simulink model "Boeing787_debug"  (R2015b)
(part 6 of 17)

      |             fcn1  = 'u(1)/39.37008' ;
      |         case 'Feet'
      |             name1 = 'ft/' ;
      |             fcn1  = 'u(1)/3.28084';
      |         case 'Yards'
      |             name1 = 'yd/' ;
      |             fcn1  = 'u(1)*3/3.28084' ;
      |         case 'Miles'
      |             name1 = 'mi/' ;
      |             fcn1  = 'u(1)*1609.344' ;
      |         case 'Nautical Miles'
      |             name1 = 'nmi/' ;
      |             fcn1  = 'u(1)*1852' ;
      |     end
      |     switch value2
      |         case 'Millisecond'
      |             name2 = 'ms' ;
      |             fcn2  = '*1000'  ;
      |         case 'Second'
      |             name2 = 's' ;
      |             fcn2  = '' ;
      |         case 'Minute'
      |             name2 = 'min' ;
      |             fcn2  = '/60' ;
      |         case 'Hour'
      |             name2 = 'hr' ;
      |             fcn2  = '/3600' ;
      |     end
      |     switch value3
      |         case 'Millimeters'
      |             name3 = 'mm/' ;
      |             fcn3  = '*1000' ;
      |         case 'Meters'
      |             name3 = 'm/' ;
      |             fcn3  = '' ;
      |         case 'Kilometers'
      |             name3 = 'km/' ;
      |             fcn3  = '/1000' ;
      |         case 'Inches'
      |             name3 = 'in/' ;
      |             fcn3  = '*39.37008' ;
      |         case 'Feet'
      |             name3 = 'ft/' ;
      |             fcn3  = '*3.28084';
      |         case 'Yards'
      |             name3 = 'yd/' ;
      |             fcn3  = '/3*3.28084' ;
      |         case 'Miles'
      |             name3 = 'mi/' ;
      |             fcn3  = '/1609.344' ;
      |         case 'Nautical Miles'
      |             name3 = 'nmi/' ;
      |             fcn3  = '/1852' ;
      |     end
      |     switch value4
      |         case 'Millisecond'
      |             name4 = 'ms' ;
      |             fcn4  = '/1000'  ;
      |         case 'Second'
      |             name4 = 's' ;
      |             fcn4  = '' ;
      |         case 'Minute'
      |             name4 = 'min' ;
      |             fcn4  = '*60' ;
      |         case 'Hour'
      |             name4 = 'hr' ;
      |             fcn4  = '*3600' ;
      |     end
      |     expr = [fcn1 fcn2 fcn3 fcn4] ;
      |     %set_param(blk,'func',func) ;
      |     set_param([blk '/conv_fcn'],'expr',expr) ;
      |     str1 = ['% this block of text is updated via dialog callbacks'];
      |     str2 = [char(39) 'horizontalAlignment' char(39) ',' char(39) 'center' char(39) ',' char(39) 'texmode' char(39) ',' char(39) 'on' char(39)] ;
      |     name = [char(39) name1 name2 ' to ' name3 name4 char(39)] ;
      |     str = sprintf('%s\ntext(.5,.5,%s,%s)',str1,name,str2) ;
      |     set_param(blk,'MaskDisplay',str) ;
      | end
      | clear blk value1 value2 value3 value4 expr name1 name2 name3 name4 name fcn1 fcn2 fcn3 fcn4 str1 str2 str
      mask TypeOptions totime: Millisecond | Second | Minute | Hour
      mask Callback totime:
      | blk = gcb ;
      | value1 = get_param(blk,'fromlen') ;
      | value2 = get_param(blk,'fromtime') ;
      | value3 = get_param(blk,'tolen') ;
      | value4 = get_param(blk,'totime') ;
      | if strcmp(get_param(blk,'vel'),'on')
      |     switch value1
      |         case 'Millimeters'
      |             name1 = 'mm/' ;
      |             fcn1  = 'u(1)/1000' ;
      |         case 'Meters'
      |             name1 = 'm/' ;
      |             fcn1  = 'u(1)' ;
      |         case 'Kilometers'
      |             name1 = 'km/' ;
      |             fcn1  = 'u(1)*1000' ;
      |         case 'Inches'
      |             name1 = 'in/' ;
      |             fcn1  = 'u(1)/39.37008' ;
      |         case 'Feet'
      |             name1 = 'ft/' ;
      |             fcn1  = 'u(1)/3.28084';
      |         case 'Yards'
      |             name1 = 'yd/' ;
      |             fcn1  = 'u(1)*3/3.28084' ;
      |         case 'Miles'
      |             name1 = 'mi/' ;
      |             fcn1  = 'u(1)*1609.344' ;
      |         case 'Nautical Miles'
      |             name1 = 'nmi/' ;
      |             fcn1  = 'u(1)*1852' ;
      |     end
      |     switch value2
      |         case 'Millisecond'
      |             name2 = 'ms' ;
      |             fcn2  = '*1000'  ;
      |         case 'Second'
      |             name2 = 's' ;
      |             fcn2  = '' ;
      |         case 'Minute'
      |             name2 = 'min' ;
      |             fcn2  = '/60' ;
      |         case 'Hour'
      |             name2 = 'hr' ;
      |             fcn2  = '/3600' ;
      |     end
      |     switch value3
      |         case 'Millimeters'
      |             name3 = 'mm/' ;
      |             fcn3  = '*1000' ;
      |         case 'Meters'
      |             name3 = 'm/' ;
      |             fcn3  = '' ;
      |         case 'Kilometers'
      |             name3 = 'km/' ;
      |             fcn3  = '/1000' ;
      |         case 'Inches'
      |             name3 = 'in/' ;
      |             fcn3  = '*39.37008' ;
      |         case 'Feet'
      |             name3 = 'ft/' ;
      |             fcn3  = '*3.28084';
      |         case 'Yards'
      |             name3 = 'yd/' ;
      |             fcn3  = '/3*3.28084' ;
      |         case 'Miles'
      |             name3 = 'mi/' ;
      |             fcn3  = '/1609.344' ;
      |         case 'Nautical Miles'
      |             name3 = 'nmi/' ;
      |             fcn3  = '/1852' ;
      |     end
      |     switch value4
      |         case 'Millisecond'
      |             name4 = 'ms' ;
      |             fcn4  = '/1000'  ;
      |         case 'Second'
      |             name4 = 's' ;
      |             fcn4  = '' ;
      |         case 'Minute'
      |             name4 = 'min' ;
      |             fcn4  = '*60' ;
      |         case 'Hour'
      |             name4 = 'hr' ;
      |             fcn4  = '*3600' ;
      |     end
      |     expr = [fcn1 fcn2 fcn3 fcn4] ;
      |     %set_param(blk,'func',func) ;
      |     set_param([blk '/conv_fcn'],'expr',expr) ;
      |     str1 = ['% this block of text is updated via dialog callbacks'];
      |     str2 = [char(39) 'horizontalAlignment' char(39) ',' char(39) 'center' char(39) ',' char(39) 'texmode' char(39) ',' char(39) 'on' char(39)] ;
      |     name = [char(39) name1 name2 ' to ' name3 name4 char(39)] ;
      |     str = sprintf('%s\ntext(.5,.5,%s,%s)',str1,name,str2) ;
      |     set_param(blk,'MaskDisplay',str) ;
      | end
      | clear blk value1 value2 value3 value4 expr name1 name2 name3 name4 name fcn1 fcn2 fcn3 fcn4 str1 str2 str
      mask Callback flow_rate:
      | blk = gcb ;
      | value = get_param(blk,'flow_rate') ;
      | cellarr = get_param(blk,'MaskVisibilities') ;
      | ind = [1 4 9 12 15 18 21 24 27 30 33 38 43] ;
      | if strcmp(value,'on')
      |     cellarr(ind) = {'off'} ; cellarr(38:42) = {'on'} ;
      |     value1 = get_param(blk,'fromflowvol') ;
      |     value2 = get_param(blk,'fromflvoltime') ;
      |     value3 = get_param(blk,'toflowvol') ;
      |     value4 = get_param(blk,'toflvoltime') ;
      |     if strcmp(get_param(blk,'flow_rate'),'on')
      |         switch value1
      |             case 'Milliliters'
      |                 name1 = 'mL/' ;
      |                 fcn1  = 'u(1)*(1e-6)' ;
      |             case 'Liters'
      |                 name1 = 'L/' ;
      |                 fcn1  = 'u(1)*.001' ;
      |             case 'Cubic Centimeters'
      |                 name1 = 'cm^3/' ;
      |                 fcn1  = 'u(1)*(1e-6)' ;
      |             case 'Cubic Meters'
      |                 name1 = 'm^3/' ;
      |                 fcn1  = 'u(1)' ;
      |             case 'Ounces'
      |                 name1 = 'oz/' ;
      |                 fcn1  = 'u(1)*(2.957353e-5)';
      |             case 'Gallons'
      |                 name1 = 'gal/' ;
      |                 fcn1  = 'u(1)*.00378541' ;
      |             case 'Cubic Inches'
      |                 name1 = 'in^3/' ;
      |                 fcn1  = 'u(1)*(1.6387e-5)' ;
      |             case 'Cubic Feet'
      |                 name1 = 'ft^3/' ;
      |                 fcn1  = 'u(1)*.0283168' ;
      |         end
      |         switch value2
      |             case 'Millisecond'
      |                 name2 = 'ms' ;
      |                 fcn2  = '*1000'  ;
      |             case 'Second'
      |                 name2 = 's' ;
      |                 fcn2  = '' ;
      |             case 'Minute'
      |                 name2 = 'min' ;
      |                 fcn2  = '/60' ;
      |             case 'Hour'
      |                 name2 = 'hr' ;
      |                 fcn2  = '/3600' ;
      |         end
      |         switch value3
      |             case 'Milliliters'
      |                 name3 = 'mL/' ;
      |                 fcn3  = '/(1e-6)' ;
      |             case 'Liters'
      |                 name3 = 'L/' ;
      |                 fcn3  = '/.001' ;
      |             case 'Cubic Centimeters'
      |                 name3 = 'cm^3/' ;
      |                 fcn3  = '/(1e-6)' ;
      |             case 'Cubic Meters'
      |                 name3 = 'm^3/' ;
      |                 fcn3  = '' ;
      |             case 'Ounces'
      |                 name3 = 'oz/' ;
      |                 fcn3  = '/(2.957353e-5)';
      |             case 'Gallons'
      |                 name3 = 'gal/' ;
      |                 fcn3  = '/.00378541' ;
      |             case 'Cubic Inches'
      |                 name3 = 'in^3/' ;
      |                 fcn3  = '/(1.6387e-5)' ;
      |             case 'Cubic Feet'
      |                 name3 = 'ft^3/' ;
      |                 fcn3  = '/.0283168' ;
      |         end
      |         switch value4
      |             case 'Millisecond'
      |                 name4 = 'ms' ;
      |                 fcn4  = '/1000'  ;
      |             case 'Second'
      |                 name4 = 's' ;
      |                 fcn4  = '' ;
      |             case 'Minute'
      |                 name4 = 'min' ;
      |                 fcn4  = '*60' ;
      |             case 'Hour'
      |                 name4 = 'hr' ;
      |                 fcn4  = '*3600' ;
      |         end
      |         expr = [fcn1 fcn2 fcn3 fcn4] ;
      |         %set_param(blk,'func',func) ;
      |         set_param([blk '/conv_fcn'],'expr',expr) ;
      |         str1 = ['% this block of text is updated via dialog callbacks'];
      |         str2 = [char(39) 'horizontalAlignment' char(39) ',' char(39) 'center' char(39) ',' char(39) 'texmode' char(39) ',' char(39) 'on' char(39)] ;
      |         name = [char(39) name1 name2 ' to ' name3 name4 char(39)] ;
      |         str = sprintf('%s\ntext(.5,.5,%s,%s)',str1,name,str2) ;
      |         set_param(blk,'MaskDisplay',str) ;
      |     end
      |     clear value1 value2 value3 value4 expr name1 name2 name3 name4 name fcn1 fcn2 fcn3 fcn4 str1 str2 str
      | else
      |     cellarr(39:42) = {'off'} ; val = get_param(blk,'MaskValues') ;
      |     for i=1:length(ind)
      |         a = findstr(val{ind(i)},'on') ;
      |         b(i) = isempty(a) ;
      |     end
      |     if isempty(find(b==0)) ;
      |         cellarr(ind) = {'on'} ;
      |     end
      | end
      | set_param(blk,'MaskVisibilities',cellarr) ;
      | clear blk value cellarr ind a b val i
      mask TypeOptions fromflowvol: Milliliters | Liters | Cubic Centimeters | Cubic Meters | Ounces | Gallons | Cubic Inches | Cubic Feet
      mask Callback fromflowvol:
      | blk = gcb ;
      | value1 = get_param(blk,'fromflowvol') ;
      | value2 = get_param(blk,'fromflvoltime') ;
      | value3 = get_param(blk,'toflowvol') ;
      | value4 = get_param(blk,'toflvoltime') ;
      | if strcmp(get_param(blk,'flow_rate'),'on')
      |     switch value1
      |         case 'Milliliters'
      |             name1 = 'mL/' ;
      |             fcn1  = 'u(1)*(1e-6)';
      |         case 'Liters'
      |             name1 = 'L/' ;
      |             fcn1  = 'u(1)*.001' ;
      |         case 'Cubic Centimeters'
      |             name1 = 'cm^3/' ;
      |             fcn1  = 'u(1)*(1e-6)' ;
      |         case 'Cubic Meters'
      |             name1 = 'm^3/' ;
      |             fcn1  = 'u(1)' ;
      |         case 'Ounces'
      |             name1 = 'oz/' ;
      |             fcn1  = 'u(1)*(2.957353e-5)';
      |         case 'Gallons'
      |             name1 = 'gal/' ;
      |             fcn1  = 'u(1)*.00378541' ;
      |         case 'Cubic Inches'
      |             name1 = 'in^3/' ;
      |             fcn1  = 'u(1)*(1.6387e-5)' ;
      |         case 'Cubic Feet'
      |             name1 = 'ft^3/' ;
      |             fcn1  = 'u(1)*.0283168' ;
      |     end
      |     switch value2
      |         case 'Millisecond'
      |             name2 = 'ms' ;
      |             fcn2  = '*1000'  ;
      |         case 'Second'
      |             name2 = 's' ;
      |             fcn2  = '' ;
      |         case 'Minute'
      |             name2 = 'min' ;
      |             fcn2  = '/60' ;
      |         case 'Hour'
      |             name2 = 'hr' ;
      |             fcn2  = '/3600' ;
      |     end
      |     switch value3
      |         case 'Milliliters'
      |             name3 = 'mL/' ;
      |             fcn3  = '/(1e-6)' ;
      |         case 'Liters'
      |             name3 = 'L/' ;
      |             fcn3  = '/.001' ;
      |         case 'Cubic Centimeters'
      |             name3 = 'cm^3/' ;
      |             fcn3  = '/(1e-6)' ;
      |         case 'Cubic Meters'
      |             name3 = 'm^3/' ;
      |             fcn3  = '' ;
      |         case 'Ounces'
      |             name3 = 'oz/' ;
      |             fcn3  = '/(2.957353e-5)';
      |         case 'Gallons'
      |             name3 = 'gal/' ;
      |             fcn3  = '/.00378541' ;
      |         case 'Cubic Inches'
      |             name3 = 'in^3/' ;
      |             fcn3  = '/(1.6387e-5)' ;
      |         case 'Cubic Feet'
      |             name3 = 'ft^3/' ;
      |             fcn3  = '/.0283168' ;
      |     end
      |     switch value4
      |         case 'Millisecond'
      |             name4 = 'ms' ;
      |             fcn4  = '/1000'  ;
      |         case 'Second'
      |             name4 = 's' ;
      |             fcn4  = '' ;
      |         case 'Minute'
      |             name4 = 'min' ;
      |             fcn4  = '*60' ;
      |         case 'Hour'
      |             name4 = 'hr' ;
      |             fcn4  = '*3600' ;
      |     end
      |     expr = [fcn1 fcn2 fcn3 fcn4] ;
      |     %set_param(blk,'func',func) ;
      |     set_param([blk '/conv_fcn'],'expr',expr) ;
      |     str1 = ['% this block of text is updated via dialog callbacks'];
      |     str2 = [char(39) 'horizontalAlignment' char(39) ',' char(39) 'center' char(39) ',' char(39) 'texmode' char(39) ',' char(39) 'on' char(39)] ;
      |     name = [char(39) name1 name2 ' to ' name3 name4 char(39)] ;
      |     str = sprintf('%s\ntext(.5,.5,%s,%s)',str1,name,str2) ;
      |     set_param(blk,'MaskDisplay',str) ;
      | end
      | clear blk value1 value2 value3 value4 expr name1 name2 name3 name4 name fcn1 fcn2 fcn3 fcn4 str1 str2 str
      mask TypeOptions fromflvoltime: Millisecond | Second | Minute | Hour
      mask Callback fromflvoltime:
      | blk = gcb ;
      | value1 = get_param(blk,'fromflowvol') ;
      | value2 = get_param(blk,'fromflvoltime') ;
      | value3 = get_param(blk,'toflowvol') ;
      | value4 = get_param(blk,'toflvoltime') ;
      | if strcmp(get_param(blk,'flow_rate'),'on')
      |     switch value1
      |         case 'Milliliters'
      |             name1 = 'mL/' ;
      |             fcn1  = 'u(1)*(1e-6)' ;
      |         case 'Liters'
      |             name1 = 'L/' ;
      |             fcn1  = 'u(1)*.001' ;
      |         case 'Cubic Centimeters'
      |             name1 = 'cm^3/' ;
      |             fcn1  = 'u(1)*(1e-6)' ;
      |         case 'Cubic Meters'
      |             name1 = 'm^3/' ;
      |             fcn1  = 'u(1)' ;
      |         case 'Ounces'
      |             name1 = 'oz/' ;
      |             fcn1  = 'u(1)*(2.957353e-5)';
      |         case 'Gallons'
      |             name1 = 'gal/' ;
      |             fcn1  = 'u(1)*.00378541' ;
      |         case 'Cubic Inches'
      |             name1 = 'in^3/' ;
      |             fcn1  = 'u(1)*(1.6387e-5)' ;
      |         case 'Cubic Feet'
      |             name1 = 'ft^3/' ;
      |             fcn1  = 'u(1)*.0283168' ;
      |     end
      |     switch value2
      |         case 'Millisecond'
      |             name2 = 'ms' ;
      |             fcn2  = '*1000'  ;
      |         case 'Second'
      |             name2 = 's' ;
      |             fcn2  = '' ;
      |         case 'Minute'
      |             name2 = 'min' ;
      |             fcn2  = '/60' ;
      |         case 'Hour'
      |             name2 = 'hr' ;
      |             fcn2  = '/3600' ;
      |     end
      |     switch value3
      |         case 'Milliliters'
      |             name3 = 'mL/' ;
      |             fcn3  = '/(1e-6)' ;
      |         case 'Liters'
      |             name3 = 'L/' ;
      |             fcn3  = '/.001' ;
      |         case 'Cubic Centimeters'
      |             name3 = 'cm^3/' ;
      |             fcn3  = '/(1e-6)' ;
      |         case 'Cubic Meters'
      |             name3 = 'm^3/' ;
      |             fcn3  = '' ;
      |         case 'Ounces'
      |             name3 = 'oz/' ;
      |             fcn3  = '/(2.957353e-5)';
      |         case 'Gallons'
      |             name3 = 'gal/' ;
      |             fcn3  = '/.00378541' ;
      |         case 'Cubic Inches'
      |             name3 = 'in^3/' ;
      |             fcn3  = '/(1.6387e-5)' ;
      |         case 'Cubic Feet'
      |             name3 = 'ft^3/' ;
      |             fcn3  = '/.0283168' ;
      |     end
      |     switch value4
      |         case 'Millisecond'
      |             name4 = 'ms' ;
      |             fcn4  = '/1000'  ;
      |         case 'Second'
      |             name4 = 's' ;
      |             fcn4  = '' ;
      |         case 'Minute'
      |             name4 = 'min' ;
      |             fcn4  = '*60' ;
      |         case 'Hour'
      |             name4 = 'hr' ;
      |             fcn4  = '*3600' ;
      |     end
      |     expr = [fcn1 fcn2 fcn3 fcn4] ;
      |     %set_param(blk,'func',func) ;
      |     set_param([blk '/conv_fcn'],'expr',expr) ;
      |     str1 = ['% this block of text is updated via dialog callbacks'];
      |     str2 = [char(39) 'horizontalAlignment' char(39) ',' char(39) 'center' char(39) ',' char(39) 'texmode' char(39) ',' char(39) 'on' char(39)] ;
      |     name = [char(39) name1 name2 ' to ' name3 name4 char(39)] ;
      |     str = sprintf('%s\ntext(.5,.5,%s,%s)',str1,name,str2) ;
      |     set_param(blk,'MaskDisplay',str) ;
      | end
      | clear blk value1 value2 value3 value4 expr name1 name2 name3 name4 name fcn1 fcn2 fcn3 fcn4 str1 str2 str
      mask TypeOptions toflowvol: Milliliters | Liters | Cubic Centimeters | Cubic Meters | Ounces | Gallons | Cubic Inches | Cubic Feet
      mask Callback toflowvol:
      | blk = gcb ;
      | value1 = get_param(blk,'fromflowvol') ;
      | value2 = get_param(blk,'fromflvoltime') ;
      | value3 = get_param(blk,'toflowvol') ;
      | value4 = get_param(blk,'toflvoltime') ;
      | if strcmp(get_param(blk,'flow_rate'),'on')
      |     switch value1
      |         case 'Milliliters'
      |             name1 = 'mL/' ;
      |             fcn1  = 'u(1)*(1e-6)' ;
      |         case 'Liters'
      |             name1 = 'L/' ;
      |             fcn1  = 'u(1)*.001' ;
      |         case 'Cubic Centimeters'
      |             name1 = 'cm^3/' ;
      |             fcn1  = 'u(1)*(1e-6)' ;
      |         case 'Cubic Meters'
      |             name1 = 'm^3/' ;
      |             fcn1  = 'u(1)' ;
      |         case 'Ounces'
      |             name1 = 'oz/' ;
      |             fcn1  = 'u(1)*(2.957353e-5)';
      |         case 'Gallons'
      |             name1 = 'gal/' ;
      |             fcn1  = 'u(1)*.00378541' ;
      |         case 'Cubic Inches'
      |             name1 = 'in^3/' ;
      |             fcn1  = 'u(1)*(1.6387e-5)' ;
      |         case 'Cubic Feet'
      |             name1 = 'ft^3/' ;
      |             fcn1  = 'u(1)*.0283168' ;
      |     end
      |     switch value2
      |         case 'Millisecond'
      |             name2 = 'ms' ;
      |             fcn2  = '*1000'  ;
      |         case 'Second'
      |             name2 = 's' ;
      |             fcn2  = '' ;
      |         case 'Minute'
      |             name2 = 'min' ;
      |             fcn2  = '/60' ;
      |         case 'Hour'
      |             name2 = 'hr' ;
      |             fcn2  = '/3600' ;
      |     end
      |     switch value3
      |         case 'Milliliters'
      |             name3 = 'mL/' ;
      |             fcn3  = '/(1e-6)' ;
      |         case 'Liters'
      |             name3 = 'L/' ;
      |             fcn3  = '/.001' ;
      |         case 'Cubic Centimeters'
      |             name3 = 'cm^3/' ;
      |             fcn3  = '/(1e-6)' ;
      |         case 'Cubic Meters'
      |             name3 = 'm^3/' ;
      |             fcn3  = '' ;
      |         case 'Ounces'
      |             name3 = 'oz/' ;
      |             fcn3  = '/(2.957353e-5)';
      |         case 'Gallons'
      |             name3 = 'gal/' ;
      |             fcn3  = '/.00378541' ;
      |         case 'Cubic Inches'
      |             name3 = 'in^3/' ;
      |             fcn3  = '/(1.6387e-5)' ;
      |         case 'Cubic Feet'
      |             name3 = 'ft^3/' ;
      |             fcn3  = '/.0283168' ;
      |     end
      |     switch value4
      |         case 'Millisecond'
      |             name4 = 'ms' ;
      |             fcn4  = '/1000'  ;
      |         case 'Second'
      |             name4 = 's' ;
      |             fcn4  = '' ;
      |         case 'Minute'
      |             name4 = 'min' ;
      |             fcn4  = '*60' ;
      |         case 'Hour'
      |             name4 = 'hr' ;
      |             fcn4  = '*3600' ;
      |     end
      |     expr = [fcn1 fcn2 fcn3 fcn4] ;
      |     %set_param(blk,'func',func) ;
      |     set_param([blk '/conv_fcn'],'expr',expr) ;
      |     str1 = ['% this block of text is updated via dialog callbacks'];
      |     str2 = [char(39) 'horizontalAlignment' char(39) ',' char(39) 'center' char(39) ',' char(39) 'texmode' char(39) ',' char(39) 'on' char(39)] ;
      |     name = [char(39) name1 name2 ' to ' name3 name4 char(39)] ;
      |     str = sprintf('%s\ntext(.5,.5,%s,%s)',str1,name,str2) ;
      |     set_param(blk,'MaskDisplay',str) ;
      | end
      | clear blk value1 value2 value3 value4 expr name1 name2 name3 name4 name fcn1 fcn2 fcn3 fcn4 str1 str2 str
      mask TypeOptions toflvoltime: Millisecond | Second | Minute | Hour
      mask Callback toflvoltime:
      | blk = gcb ;
      | value1 = get_param(blk,'fromflowvol') ;
      | value2 = get_param(blk,'fromflvoltime') ;
      | value3 = get_param(blk,'toflowvol') ;
      | value4 = get_param(blk,'toflvoltime') ;
      | if strcmp(get_param(blk,'flow_rate'),'on')
      |     switch value1
      |         case 'Milliliters'
      |             name1 = 'mL/' ;
      |             fcn1  = 'u(1)*(1e-6)' ;
      |         case 'Liters'
      |             name1 = 'L/' ;
      |             fcn1  = 'u(1)*.001' ;
      |         case 'Cubic Centimeters'
      |             name1 = 'cm^3/' ;
      |             fcn1  = 'u(1)*(1e-6)' ;
      |         case 'Cubic Meters'
      |             name1 = 'm^3/' ;
      |             fcn1  = 'u(1)' ;
      |         case 'Ounces'
      |             name1 = 'oz/' ;
      |             fcn1  = 'u(1)*(2.957353e-5)';
      |         case 'Gallons'
      |             name1 = 'gal/' ;
      |             fcn1  = 'u(1)*.00378541' ;
      |         case 'Cubic Inches'
      |             name1 = 'in^3/' ;
      |             fcn1  = 'u(1)*(1.6387e-5)' ;
      |         case 'Cubic Feet'
      |             name1 = 'ft^3/' ;
      |             fcn1  = 'u(1)*.0283168' ;
      |     end
      |     switch value2
      |         case 'Millisecond'
      |             name2 = 'ms' ;
      |             fcn2  = '*1000'  ;
      |         case 'Second'
      |             name2 = 's' ;
      |             fcn2  = '' ;
      |         case 'Minute'
      |             name2 = 'min' ;
      |             fcn2  = '/60' ;
      |         case 'Hour'
      |             name2 = 'hr' ;
      |             fcn2  = '/3600' ;
      |     end
      |     switch value3
      |         case 'Milliliters'
      |             name3 = 'mL/' ;
      |             fcn3  = '/(1e-6)' ;
      |         case 'Liters'
      |             name3 = 'L/' ;
      |             fcn3  = '/.001' ;
      |         case 'Cubic Centimeters'
      |             name3 = 'cm^3/' ;
      |             fcn3  = '/(1e-6)' ;
      |         case 'Cubic Meters'
      |             name3 = 'm^3/' ;
      |             fcn3  = '' ;
      |         case 'Ounces'
      |             name3 = 'oz/' ;
      |             fcn3  = '/(2.957353e-5)';
      |         case 'Gallons'
      |             name3 = 'gal/' ;
      |             fcn3  = '/.00378541' ;
      |         case 'Cubic Inches'
      |             name3 = 'in^3/' ;
      |             fcn3  = '/(1.6387e-5)' ;
      |         case 'Cubic Feet'
      |             name3 = 'ft^3/' ;
      |             fcn3  = '/.0283168' ;
      |     end
      |     switch value4
      |         case 'Millisecond'
      |             name4 = 'ms' ;
      |             fcn4  = '/1000'  ;
      |         case 'Second'
      |             name4 = 's' ;
      |             fcn4  = '' ;
      |         case 'Minute'
      |             name4 = 'min' ;
      |             fcn4  = '*60' ;
      |         case 'Hour'
      |             name4 = 'hr' ;
      |             fcn4  = '*3600' ;
      |     end
      |     expr = [fcn1 fcn2 fcn3 fcn4] ;
      |     %set_param(blk,'func',func) ;
      |     set_param([blk '/conv_fcn'],'expr',expr) ;
      |     str1 = ['% this block of text is updated via dialog callbacks'];
      |     str2 = [char(39) 'horizontalAlignment' char(39) ',' char(39) 'center' char(39) ',' char(39) 'texmode' char(39) ',' char(39) 'on' char(39)] ;
      |     name = [char(39) name1 name2 ' to ' name3 name4 char(39)] ;
      |     str = sprintf('%s\ntext(.5,.5,%s,%s)',str1,name,str2) ;
      |     set_param(blk,'MaskDisplay',str) ;
      | end
      | clear blk value1 value2 value3 value4 expr name1 name2 name3 name4 name fcn1 fcn2 fcn3 fcn4 str1 str2 str
      mask Callback mfr:
      | blk = gcb ;
      | value = get_param(blk,'mfr') ;
      | cellarr = get_param(blk,'MaskVisibilities') ;
      | ind = [1 4 9 12 15 18 21 24 27 30 33 38 43] ;
      | if strcmp(value,'on')
      |     cellarr(ind) = {'off'} ; cellarr(43:47) = {'on'} ;
      |     value1 = get_param(blk,'frommfr') ;
      |     value2 = get_param(blk,'frommfrtime') ;
      |     value3 = get_param(blk,'tomfr') ;
      |     value4 = get_param(blk,'tomfrtime') ;
      |     if strcmp(get_param(blk,'mfr'),'on')
      |         switch value1
      |             case 'Grams'
      |                 name1 = 'g/' ;
      |                 fcn1  = 'u(1)*.001' ;
      |             case 'Kilograms'
      |                 name1 = 'kg/' ;
      |                 fcn1  = 'u(1)' ;
      |             case 'Ounces'
      |                 name1 = 'oz/' ;
      |                 fcn1  = 'u(1)*.45359237/16' ;
      |             case 'Pounds-Mass'
      |                 name1 = 'lbm/' ;
      |                 fcn1  = 'u(1)*.45359237' ;
      |             case 'Slugs'
      |                 name1 = 'slg/' ;
      |                 fcn1  = 'u(1)*14.5939';
      |         end
      |         switch value2
      |             case 'Millisecond'
      |                 name2 = 'ms' ;
      |                 fcn2  = '*1000'  ;
      |             case 'Second'
      |                 name2 = 's' ;
      |                 fcn2  = '' ;
      |             case 'Minute'
      |                 name2 = 'min' ;
      |                 fcn2  = '/60' ;
      |             case 'Hour'
      |                 name2 = 'hr' ;
      |                 fcn2  = '/3600' ;
      |         end
      |         switch value3
      |             case 'Grams'
      |                 name3 = 'g/' ;
      |                 fcn3  = '/.001' ;
      |             case 'Kilograms'
      |                 name3 = 'kg/' ;
      |                 fcn3  = '' ;
      |             case 'Ounces'
      |                 name3 = 'oz/' ;
      |                 fcn3  = '/.45359237*16' ;
      |             case 'Pounds-Mass'
      |                 name3 = 'lbm/' ;
      |                 fcn3  = '/.45359237' ;
      |             case 'Slugs'
      |                 name3 = 'slg/' ;
      |                 fcn3  = '/14.5939';
      |         end
      |         switch value4
      |             case 'Millisecond'
      |                 name4 = 'ms' ;
      |                 fcn4  = '/1000'  ;
      |             case 'Second'
      |                 name4 = 's' ;
      |                 fcn4  = '' ;
      |             case 'Minute'
      |                 name4 = 'min' ;
      |                 fcn4  = '*60' ;
      |             case 'Hour'
      |                 name4 = 'hr' ;
      |                 fcn4  = '*3600' ;
      |         end
      |         expr = [fcn1 fcn2 fcn3 fcn4] ;
      |         %set_param(blk,'func',func) ;
      |         set_param([blk '/conv_fcn'],'expr',expr) ;
      |         str1 = ['% this block of text is updated via dialog callbacks'];
      |         str2 = [char(39) 'horizontalAlignment' char(39) ',' char(39) 'center' char(39) ',' char(39) 'texmode' char(39) ',' char(39) 'on' char(39)] ;
      |         name = [char(39) name1 name2 ' to ' name3 name4 char(39)] ;
      |         str = sprintf('%s\ntext(.5,.5,%s,%s)',str1,name,str2) ;
      |         set_param(blk,'MaskDisplay',str) ;
      |     end
      |     clear value1 value2 value3 value4 expr name1 name2 name3 name4 name fcn1 fcn2 fcn3 fcn4 str1 str2 str
      | else
      |     cellarr(44:47) = {'off'} ; val = get_param(blk,'MaskValues') ;
      |     for i=1:length(ind)
      |         a = findstr(val{ind(i)},'on') ;
      |         b(i) = isempty(a) ;
      |     end
      |     if isempty(find(b==0)) ;
      |         cellarr(ind) = {'on'} ;
      |     end
      | end
      | set_param(blk,'MaskVisibilities',cellarr) ;
      | clear blk value cellarr ind a b val i
      mask TypeOptions frommfr: Grams | Kilograms | Ounces | Pounds-Mass | Slugs
      mask Callback frommfr:
      | blk = gcb ;
      | value1 = get_param(blk,'frommfr') ;
      | value2 = get_param(blk,'frommfrtime') ;
      | value3 = get_param(blk,'tomfr') ;
      | value4 = get_param(blk,'tomfrtime') ;
      | if strcmp(get_param(blk,'mfr'),'on')
      |     switch value1
      |         case 'Grams'
      |             name1 = 'g/' ;
      |             fcn1  = 'u(1)*.001' ;
      |         case 'Kilograms'
      |             name1 = 'kg/' ;
      |             fcn1  = 'u(1)' ;
      |         case 'Ounces'
      |             name1 = 'oz/' ;
      |             fcn1  = 'u(1)*.45359237/16' ;
      |         case 'Pounds-Mass'
      |             name1 = 'lbm/' ;
      |             fcn1  = 'u(1)*.45359237' ;
      |         case 'Slugs'
      |             name1 = 'slg/' ;
      |             fcn1  = 'u(1)*14.5939';
      |     end
      |     switch value2
      |         case 'Millisecond'
      |             name2 = 'ms' ;
      |             fcn2  = '*1000'  ;
      |         case 'Second'
      |             name2 = 's' ;
      |             fcn2  = '' ;
      |         case 'Minute'
      |             name2 = 'min' ;
      |             fcn2  = '/60' ;
      |         case 'Hour'
      |             name2 = 'hr' ;
      |             fcn2  = '/3600' ;
      |     end
      |     switch value3
      |         case 'Grams'
      |             name3 = 'g/' ;
      |             fcn3  = '/.001' ;
      |         case 'Kilograms'
      |             name3 = 'kg/' ;
      |             fcn3  = '' ;
      |         case 'Ounces'
      |             name3 = 'oz/' ;
      |             fcn3  = '/.45359237*16' ;
      |         case 'Pounds-Mass'
      |             name3 = 'lbm/' ;
      |             fcn3  = '/.45359237' ;
      |         case 'Slugs'
      |             name3 = 'slg/' ;
      |             fcn3  = '/14.5939';
      |     end
      |     switch value4
      |         case 'Millisecond'
      |             name4 = 'ms' ;
      |             fcn4  = '/1000'  ;
      |         case 'Second'
      |             name4 = 's' ;
      |             fcn4  = '' ;
      |         case 'Minute'
      |             name4 = 'min' ;
      |             fcn4  = '*60' ;
      |         case 'Hour'
      |             name4 = 'hr' ;
      |             fcn4  = '*3600' ;
      |     end
      |     expr = [fcn1 fcn2 fcn3 fcn4] ;
      |     %set_param(blk,'func',func) ;
      |     set_param([blk '/conv_fcn'],'expr',expr) ;
      |     str1 = ['% this block of text is updated via dialog callbacks'];
      |     str2 = [char(39) 'horizontalAlignment' char(39) ',' char(39) 'center' char(39) ',' char(39) 'texmode' char(39) ',' char(39) 'on' char(39)] ;
      |     name = [char(39) name1 name2 ' to ' name3 name4 char(39)] ;
      |     str = sprintf('%s\ntext(.5,.5,%s,%s)',str1,name,str2) ;
      |     set_param(blk,'MaskDisplay',str) ;
      | end
      | clear blk value1 value2 value3 value4 expr name1 name2 name3 name4 name fcn1 fcn2 fcn3 fcn4 str1 str2 str
      mask TypeOptions frommfrtime: Millisecond | Second | Minute | Hour
      mask Callback frommfrtime:
      | blk = gcb ;
      | value1 = get_param(blk,'frommfr') ;
      | value2 = get_param(blk,'frommfrtime') ;
      | value3 = get_param(blk,'tomfr') ;
      | value4 = get_param(blk,'tomfrtime') ;
      | if strcmp(get_param(blk,'mfr'),'on')
      |     switch value1
      |         case 'Grams'
      |             name1 = 'g/' ;
      |             fcn1  = 'u(1)*.001' ;
      |         case 'Kilograms'
      |             name1 = 'kg/' ;
      |             fcn1  = 'u(1)' ;
      |         case 'Ounces'
      |             name1 = 'oz/' ;
      |             fcn1  = 'u(1)*.45359237/16' ;
      |         case 'Pounds-Mass'
      |             name1 = 'lbm/' ;
      |             fcn1  = 'u(1)*.45359237' ;
      |         case 'Slugs'
      |             name1 = 'slg/' ;
      |             fcn1  = 'u(1)*14.5939';
      |     end
      |     switch value2
      |         case 'Millisecond'
      |             name2 = 'ms' ;
      |             fcn2  = '*1000'  ;
      |         case 'Second'
      |             name2 = 's' ;
      |             fcn2  = '' ;
      |         case 'Minute'
      |             name2 = 'min' ;
      |             fcn2  = '/60' ;
      |         case 'Hour'
      |             name2 = 'hr' ;
      |             fcn2  = '/3600' ;
      |     end
      |     switch value3
      |         case 'Grams'
      |             name3 = 'g/' ;
      |             fcn3  = '/.001' ;
      |         case 'Kilograms'
      |             name3 = 'kg/' ;
      |             fcn3  = '' ;
      |         case 'Ounces'
      |             name3 = 'oz/' ;
      |             fcn3  = '/.45359237*16' ;
      |         case 'Pounds-Mass'
      |             name3 = 'lbm/' ;
      |             fcn3  = '/.45359237' ;
      |         case 'Slugs'
      |             name3 = 'slg/' ;
      |             fcn3  = '/14.5939';
      |     end
      |     switch value4
      |         case 'Millisecond'
      |             name4 = 'ms' ;
      |             fcn4  = '/1000'  ;
      |         case 'Second'
      |             name4 = 's' ;
      |             fcn4  = '' ;
      |         case 'Minute'
      |             name4 = 'min' ;
      |             fcn4  = '*60' ;
      |         case 'Hour'
      |             name4 = 'hr' ;
      |             fcn4  = '*3600' ;
      |     end
      |     expr = [fcn1 fcn2 fcn3 fcn4] ;
      |     %set_param(blk,'func',func) ;
      |     set_param([blk '/conv_fcn'],'expr',expr) ;
      |     str1 = ['% this block of text is updated via dialog callbacks'];
      |     str2 = [char(39) 'horizontalAlignment' char(39) ',' char(39) 'center' char(39) ',' char(39) 'texmode' char(39) ',' char(39) 'on' char(39)] ;
      |     name = [char(39) name1 name2 ' to ' name3 name4 char(39)] ;
      |     str = sprintf('%s\ntext(.5,.5,%s,%s)',str1,name,str2) ;
      |     set_param(blk,'MaskDisplay',str) ;
      | end
      | clear blk value1 value2 value3 value4 expr name1 name2 name3 name4 name fcn1 fcn2 fcn3 fcn4 str1 str2 str
      mask TypeOptions tomfr: Grams | Kilograms | Ounces | Pounds-Mass | Slugs
      mask Callback tomfr:
      | blk = gcb ;
      | value1 = get_param(blk,'frommfr') ;
      | value2 = get_param(blk,'frommfrtime') ;
      | value3 = get_param(blk,'tomfr') ;
      | value4 = get_param(blk,'tomfrtime') ;
      | if strcmp(get_param(blk,'mfr'),'on')
      |     switch value1
      |         case 'Grams'
      |             name1 = 'g/' ;
      |             fcn1  = 'u(1)*.001' ;
      |         case 'Kilograms'
      |             name1 = 'kg/' ;
      |             fcn1  = 'u(1)' ;
      |         case 'Ounces'
      |             name1 = 'oz/' ;
      |             fcn1  = 'u(1)*.45359237/16' ;
      |         case 'Pounds-Mass'
      |             name1 = 'lbm/' ;
      |             fcn1  = 'u(1)*.45359237' ;
      |         case 'Slugs'
      |             name1 = 'slg/' ;
      |             fcn1  = 'u(1)*14.5939';
      |     end
      |     switch value2
      |         case 'Millisecond'
      |             name2 = 'ms' ;
      |             fcn2  = '*1000'  ;
      |         case 'Second'
      |             name2 = 's' ;
      |             fcn2  = '' ;
      |         case 'Minute'
      |             name2 = 'min' ;
      |             fcn2  = '/60' ;
      |         case 'Hour'
      |             name2 = 'hr' ;
      |             fcn2  = '/3600' ;
      |     end
      |     switch value3
      |         case 'Grams'
      |             name3 = 'g/' ;
      |             fcn3  = '/.001' ;
      |         case 'Kilograms'
      |             name3 = 'kg/' ;
      |             fcn3  = '' ;
      |         case 'Ounces'
      |             name3 = 'oz/' ;
      |             fcn3  = '/.45359237*16' ;
      |         case 'Pounds-Mass'
      |             name3 = 'lbm/' ;
      |             fcn3  = '/.45359237' ;
      |         case 'Slugs'
      |             name3 = 'slg/' ;
      |             fcn3  = '/14.5939';
      |     end
      |     switch value4
      |         case 'Millisecond'
      |             name4 = 'ms' ;
      |             fcn4  = '/1000'  ;
      |         case 'Second'
      |             name4 = 's' ;
      |             fcn4  = '' ;
      |         case 'Minute'
      |             name4 = 'min' ;
      |             fcn4  = '*60' ;
      |         case 'Hour'
      |             name4 = 'hr' ;
      |             fcn4  = '*3600' ;
      |     end
      |     expr = [fcn1 fcn2 fcn3 fcn4] ;
      |     %set_param(blk,'func',func) ;
      |     set_param([blk '/conv_fcn'],'expr',expr) ;
      |     str1 = ['% this block of text is updated via dialog callbacks'];
      |     str2 = [char(39) 'horizontalAlignment' char(39) ',' char(39) 'center' char(39) ',' char(39) 'texmode' char(39) ',' char(39) 'on' char(39)] ;
      |     name = [char(39) name1 name2 ' to ' name3 name4 char(39)] ;
      |     str = sprintf('%s\ntext(.5,.5,%s,%s)',str1,name,str2) ;
      |     set_param(blk,'MaskDisplay',str) ;
      | end
      | clear blk value1 value2 value3 value4 expr name1 name2 name3 name4 name fcn1 fcn2 fcn3 fcn4 str1 str2 str
      mask TypeOptions tomfrtime: Millisecond | Second | Minute | Hour
      mask Callback tomfrtime:
      | blk = gcb ;
      | value1 = get_param(blk,'frommfr') ;
      | value2 = get_param(blk,'frommfrtime') ;
      | value3 = get_param(blk,'tomfr') ;
      | value4 = get_param(blk,'tomfrtime') ;
      | if strcmp(get_param(blk,'mfr'),'on')
      |     switch value1
      |         case 'Grams'
      |             name1 = 'g/' ;
      |             fcn1  = 'u(1)*.001' ;
      |         case 'Kilograms'
      |             name1 = 'kg/' ;
      |             fcn1  = 'u(1)' ;
      |         case 'Ounces'
      |             name1 = 'oz/' ;
      |             fcn1  = 'u(1)*.45359237/16' ;
      |         case 'Pounds-Mass'
      |             name1 = 'lbm/' ;
      |             fcn1  = 'u(1)*.45359237' ;
      |         case 'Slugs'
      |             name1 = 'slg/' ;
      |             fcn1  = 'u(1)*14.5939';
      |     end
      |     switch value2
      |         case 'Millisecond'
      |             name2 = 'ms' ;
      |             fcn2  = '*1000'  ;
      |         case 'Second'
      |             name2 = 's' ;
      |             fcn2  = '' ;
      |         case 'Minute'
      |             name2 = 'min' ;
      |             fcn2  = '/60' ;
      |         case 'Hour'
      |             name2 = 'hr' ;
      |             fcn2  = '/3600' ;
      |     end
      |     switch value3
      |         case 'Grams'
      |             name3 = 'g/' ;
      |             fcn3  = '/.001' ;
      |         case 'Kilograms'
      |             name3 = 'kg/' ;
      |             fcn3  = '' ;
      |         case 'Ounces'
      |             name3 = 'oz/' ;
      |             fcn3  = '/.45359237*16' ;
      |         case 'Pounds-Mass'
      |             name3 = 'lbm/' ;
      |             fcn3  = '/.45359237' ;
      |         case 'Slugs'
      |             name3 = 'slg/' ;
      |             fcn3  = '/14.5939';
      |     end
      |     switch value4
      |         case 'Millisecond'
      |             name4 = 'ms' ;
      |             fcn4  = '/1000'  ;
      |         case 'Second'
      |             name4 = 's' ;
      |             fcn4  = '' ;
      |         case 'Minute'
      |             name4 = 'min' ;
      |             fcn4  = '*60' ;
      |         case 'Hour'
      |             name4 = 'hr' ;
      |             fcn4  = '*3600' ;
      |     end
      |     expr = [fcn1 fcn2 fcn3 fcn4] ;
      |     %set_param(blk,'func',func) ;
      |     set_param([blk '/conv_fcn'],'expr',expr) ;
      |     str1 = ['% this block of text is updated via dialog callbacks'];
      |     str2 = [char(39) 'horizontalAlignment' char(39) ',' char(39) 'center' char(39) ',' char(39) 'texmode' char(39) ',' char(39) 'on' char(39)] ;
      |     name = [char(39) name1 name2 ' to ' name3 name4 char(39)] ;
      |     str = sprintf('%s\ntext(.5,.5,%s,%s)',str1,name,str2) ;
      |     set_param(blk,'MaskDisplay',str) ;
      | end
      | clear blk value1 value2 value3 value4 expr name1 name2 name3 name4 name fcn1 fcn2 fcn3 fcn4 str1 str2 str
      mask Display:
      | % this block of text is updated via dialog callbacks
      | text(.5,.5,'psia to kPa','horizontalAlignment','center','texmode','on')
  Unit Conversion 5 : Subsystem  mask(Unit conversion){mass=off, frommass=Grams, tomass=Pounds-Mass, dens=off, fromdens=Pounds-Mass, perdens=Cubic Feet, todens=Kilograms, toperdens=Cubic Meters, energy=off, fromenergy=Joules, toenergy=Joules, power=off, frompower=Watts, topower=Horsepower, force=off, fromforce=Newtons, toforce=Newtons, temp=off, fromtemp=Celcius, totemp=Celcius, pres=off, frompres=psia, topres=psia, length=off, fromlength=Millimeters, tolength=Millimeters, area=off, fromarea=Square Centimeters, toarea=Square Centimeters, vol=off, fromvol=Milliliters, tovol=Milliliters, vel=off, fromlen=Millimeters, fromtime=Millisecond, tolen=Millimeters, totime=Millisecond, flow_rate=off, fromflowvol=Milliliters, fromflvoltime=Millisecond, toflowvol=Milliliters, toflvoltime=Millisecond, mfr=on, frommfr=Pounds-Mass, frommfrtime=Second, tomfr=Kilograms, tomfrtime=Second}
      mask prompts: frommass "From :"; tomass "To :"; dens "Density"; fromdens "From :"; perdens "per"; todens "To :"; toperdens "per"; fromenergy "From :"; toenergy "To :"; frompower "From :"; topower "To :"; fromforce "From :"; toforce "To :"; temp "Temperature"; fromtemp "From :"; totemp "To :"; pres "Pressure"; frompres "From :"; topres "To :"; fromlength "From :"; tolength "To :"; fromarea "From :"; toarea "To :"; vol "Volume"; fromvol "From :"; tovol "To :"; vel "Velocity"; fromlen "From :........."; fromtime "per"; tolen "To :.........."; totime "per"; flow_rate "Volume Flow Rate"; fromflowvol "From :........."; fromflvoltime "per"; toflowvol "To :.........."; toflvoltime "per"; mfr "Mass Flow Rate"; frommfr "From :........."; frommfrtime "per"; tomfr "To :.........."; tomfrtime "per"
      mask help:
      | Convert units of:
      |
      | Mass, density, energy, power, force, temperature, pressure, length, area, volume, velocity, and flow rate
      mask init: same as Boeing787_debug/Eng1/Unit Conversion 
      mask Callback mass:
      | blk = gcb ;
      | value = get_param(blk,'mass') ;
      | cellarr = get_param(blk,'MaskVisibilities') ;
      | ind = [1 4 9 12 15 18 21 24 27 30 33 38 43] ;
      | if strcmp(value,'on')
      |     cellarr(ind) = {'off'} ; cellarr(1:3) = {'on'} ;
      |     value1 = get_param(blk,'frommass') ;
      |     value2 = get_param(blk,'tomass') ;
      |     if strcmp(get_param(blk,'mass'),'on') ;
      |         switch value1
      |             case 'Grams'
      |                 name1 = 'gr' ;
      |                 fcn1  = 'u(1)*.001' ;
      |             case 'Kilograms'
      |                 name1 = 'kg' ;
      |                 fcn1  = 'u(1)' ;
      |             case 'Ounces'
      |                 name1 = 'oz' ;
      |                 fcn1  = 'u(1)*.45359237/16' ;
      |             case 'Pounds-Mass'
      |                 name1 = 'lbm' ;
      |                 fcn1  = 'u(1)*.45359237' ;
      |             case 'Slugs'
      |                 name1 = 'slg' ;
      |                 fcn1  = 'u(1)*14.5939029' ;
      |         end
      |         switch value2
      |             case 'Grams'
      |                 name2 = 'gr' ;
      |                 fcn2  = '/.001' ;
      |             case 'Kilograms'
      |                 name2 = 'kg' ;
      |                 fcn2  = '' ;
      |             case 'Ounces'
      |                 name2 = 'oz' ;
      |                 fcn2  = '/.45359237*16' ;
      |             case 'Pounds-Mass'
      |                 name2 = 'lbm' ;
      |                 fcn2  = '/.45359237' ;
      |             case 'Slugs'
      |                 name2 = 'slg' ;
      |                 fcn2  = '/14.5939029' ;
      |         end
      |         expr = [fcn1 fcn2] ;
      |         %set_param(blk,'func',func) ;
      |         set_param([blk '/conv_fcn'],'expr',expr) ;
      |         str1 = ['% this block of text is updated via dialog callbacks'];
      |         str2 = [char(39) 'horizontalAlignment' char(39) ',' char(39) 'center' char(39) ',' char(39) 'texmode' char(39) ',' char(39) 'on' char(39)] ;
      |         name = [char(39) name1 ' to ' name2 char(39)] ;
      |         str = sprintf('%s\ntext(.5,.5,%s,%s)',str1,name,str2) ;
      |         set_param(blk,'MaskDisplay',str) ;
      |     end
      |     clear value1 value2 expr name1 name2 name fcn1 fcn2 str1 str2 str
      | else
      |     cellarr(2:3) = {'off'} ; val = get_param(blk,'MaskValues') ;
      |     for i=1:length(ind)
      |         a = findstr(val{ind(i)},'on') ;
      |         b(i) = isempty(a) ;
      |     end
      |     if isempty(find(b==0)) ;
      |         cellarr(ind) = {'on'} ;
      |     end
      | end
      | set_param(blk,'MaskVisibilities',cellarr) ;
      | clear blk value cellarr ind a b val i
      mask TypeOptions frommass: Grams | Kilograms | Ounces | Pounds-Mass | Slugs
      mask Callback frommass:
      | blk = gcb ;
      | value1 = get_param(blk,'frommass') ;
      | value2 = get_param(blk,'tomass') ;
      | if strcmp(get_param(blk,'mass'),'on') ;
      |     switch value1
      |         case 'Grams'
      |             name1 = 'gr' ;
      |             fcn1  = 'u(1)*.001' ;
      |         case 'Kilograms'
      |             name1 = 'kg' ;
      |             fcn1  = 'u(1)' ;
      |         case 'Ounces'
      |             name1 = 'oz' ;
      |             fcn1  = 'u(1)*.45359237/16' ;
      |         case 'Pounds-Mass'
      |             name1 = 'lbm' ;
      |             fcn1  = 'u(1)*.45359237' ;
      |         case 'Slugs'
      |             name1 = 'slg' ;
      |             fcn1  = 'u(1)*14.5939029' ;
      |     end
      |     switch value2
      |         case 'Grams'
      |             name2 = 'gr' ;
      |             fcn2  = '/.001' ;
      |         case 'Kilograms'
      |             name2 = 'kg' ;
      |             fcn2  = '' ;
      |         case 'Ounces'
      |             name2 = 'oz' ;
      |             fcn2  = '/.45359237*16' ;
      |         case 'Pounds-Mass'
      |             name2 = 'lbm' ;
      |             fcn2  = '/.45359237' ;
      |         case 'Slugs'
      |             name2 = 'slg' ;
      |             fcn2  = '/14.5939029' ;
      |     end
      |     expr = [fcn1 fcn2] ;
      |     %set_param(blk,'func',func) ;
      |     set_param([blk '/conv_fcn'],'expr',expr) ;
      |     str1 = ['% this block of text is updated via dialog callbacks'];
      |         str2 = [char(39) 'horizontalAlignment' char(39) ',' char(39) 'center' char(39) ',' char(39) 'texmode' char(39) ',' char(39) 'on' char(39)] ;
      |     name = [char(39) name1 ' to ' name2 char(39)] ;
      |     str = sprintf('%s\ntext(.5,.5,%s,%s)',str1,name,str2) ;
      |     set_param(blk,'MaskDisplay',str) ;
      | end
      |     clear blk value1 value2 expr name1 name2 name fcn1 fcn2 str1 str2 str
      mask TypeOptions tomass: Grams | Kilograms | Ounces | Pounds-Mass | Slugs
      mask Callback tomass:
      | blk = gcb ;
      | value1 = get_param(blk,'frommass') ;
      | value2 = get_param(blk,'tomass') ;
      | if strcmp(get_param(blk,'mass'),'on') ;
      |     switch value1
      |         case 'Grams'
      |             name1 = 'gr' ;
      |             fcn1  = 'u(1)*.001' ;
      |         case 'Kilograms'
      |             name1 = 'kg' ;
      |             fcn1  = 'u(1)' ;
      |         case 'Ounces'
      |             name1 = 'oz' ;
      |             fcn1  = 'u(1)*.45359237/16' ;
      |         case 'Pounds-Mass'
      |             name1 = 'lbm' ;
      |             fcn1  = 'u(1)*.45359237' ;
      |         case 'Slugs'
      |             name1 = 'slg' ;
      |             fcn1  = 'u(1)*14.5939029' ;
      |     end
      |     switch value2
      |         case 'Grams'
      |             name2 = 'gr' ;
      |             fcn2  = '/.001' ;
      |         case 'Kilograms'
      |             name2 = 'kg' ;
      |             fcn2  = '' ;
      |         case 'Ounces'
      |             name2 = 'oz' ;
      |             fcn2  = '/.45359237*16' ;
      |         case 'Pounds-Mass'
      |             name2 = 'lbm' ;
      |             fcn2  = '/.45359237' ;
      |         case 'Slugs'
      |             name2 = 'slg' ;
      |             fcn2  = '/14.5939029' ;
      |     end
      |     expr = [fcn1 fcn2] ;
      |     %set_param(blk,'func',func) ;
      |     set_param([blk '/conv_fcn'],'expr',expr) ;
      |     str1 = ['% this block of text is updated via dialog callbacks'];
      |         str2 = [char(39) 'horizontalAlignment' char(39) ',' char(39) 'center' char(39) ',' char(39) 'texmode' char(39) ',' char(39) 'on' char(39)] ;
      |     name = [char(39) name1 ' to ' name2 char(39)] ;
      |     str = sprintf('%s\ntext(.5,.5,%s,%s)',str1,name,str2) ;
      |     set_param(blk,'MaskDisplay',str) ;
      | end
      |     clear blk value1 value2 expr name1 name2 name fcn1 fcn2 str1 str2 str
      mask Callback dens:
      | blk = gcb ;
      | value = get_param(blk,'dens') ;
      | cellarr = get_param(blk,'MaskVisibilities');
      | ind = [1 4 9 12 15 18 21 24 27 30 33 38 43] ;
      | if strcmp(value,'on')
      |     cellarr(ind) = {'off'} ; cellarr(4:8) = {'on'} ;
      |     value1 = get_param(blk,'fromdens') ;
      |     value2 = get_param(blk,'perdens') ;
      |     value3 = get_param(blk,'todens') ;
      |     value4 = get_param(blk,'toperdens') ;
      |     if strcmp(get_param(blk,'dens'),'on')
      |         switch value1
      |             case 'Grams'
      |                 name1 = 'g/' ;
      |                 fcn1  = 'u(1)*.001' ;
      |             case 'Kilograms'
      |                 name1 = 'kg/' ;
      |                 fcn1  = 'u(1)' ;
      |             case 'Ounces'
      |                 name1 = 'oz/' ;
      |                 fcn1  = 'u(1)*.45359237/16' ;
      |             case 'Pounds-Mass'
      |                 name1 = 'lbm/' ;
      |                 fcn1  = 'u(1)*.45359237' ;
      |             case 'Slugs'
      |                 name1 = 'slg/' ;
      |                 fcn1  = 'u(1)*14.5939';
      |         end
      |         switch value2
      |             case 'Milliliters'
      |                 name2 = 'mL' ;
      |                 fcn2  = '/(1e-6)' ;
      |             case 'Liters'
      |                 name2 = 'L' ;
      |                 fcn2  = '/.001' ;
      |             case 'Cubic Centimeters'
      |                 name2 = 'cm^3' ;
      |                 fcn2  = '/(1e-6)' ;
      |             case 'Cubic Meters'
      |                 name2 = 'm^3' ;
      |                 fcn2  = '' ;
      |             case 'Ounces'
      |                 name2 = 'oz' ;
      |                 fcn2  = '/(2.95735e-5)' ;
      |             case 'Gallons'
      |                 name2 = 'gal' ;
      |                 fcn2  = '/.0037854' ;
      |             case 'Cubic Inches'
      |                 name2 = 'in^3' ;
      |                 fcn2  = '/(1.6387e-5)' ;
      |             case 'Cubic Feet'
      |                 name2 = 'ft^3' ;
      |                 fcn2  = '/.02831685' ;
      |         end
      |         switch value3
      |             case 'Grams'
      |                 name3 = 'g/' ;
      |                 fcn3  = '/.001' ;
      |             case 'Kilograms'
      |                 name3 = 'kg/' ;
      |                 fcn3  = '' ;
      |             case 'Ounces'
      |                 name3 = 'oz/' ;
      |                 fcn3  = '/.45359237*16' ;
      |             case 'Pounds-Mass'
      |                 name3 = 'lbm/' ;
      |                 fcn3  = '/.45359237' ;
      |             case 'Slugs'
      |                 name3 = 'slg/' ;
      |                 fcn3  = '/14.5939';
      |         end
      |         switch value4
      |             case 'Milliliters'
      |                 name4 = 'mL' ;
      |                 fcn4  = '*(1e-6)' ;
      |             case 'Liters'
      |                 name4 = 'L' ;
      |                 fcn4  = '*.001' ;
      |             case 'Cubic Centimeters'
      |                 name4 = 'cm^3' ;
      |                 fcn4  = '*(1e-6)' ;
      |             case 'Cubic Meters'
      |                 name4 = 'm^3' ;
      |                 fcn4  = '' ;
      |             case 'Ounces'
      |                 name4 = 'oz' ;
      |                 fcn4  = '*(2.95735e-5)' ;
      |             case 'Gallons'
      |                 name4 = 'gal' ;
      |                 fcn4  = '*.0037854' ;
      |             case 'Cubic Inches'
      |                 name4 = 'in^3' ;
      |                 fcn4  = '*(1.6387e-5)' ;
      |             case 'Cubic Feet'
      |                 name4 = 'ft^3' ;
      |                 fcn4  = '*.02831685' ;
      |         end
      |         expr = [fcn1 fcn2 fcn3 fcn4] ;
      |         %set_param(blk,'func',func) ;
      |         set_param([blk '/conv_fcn'],'expr',expr) ;
      |         str1 = ['% this block of text is updated via dialog callbacks'];
      |         str2 = [char(39) 'horizontalAlignment' char(39) ',' char(39) 'center' char(39) ',' char(39) 'texmode' char(39) ',' char(39) 'on' char(39)] ;
      |         name = [char(39) name1 name2 ' to ' name3 name4 char(39)] ;
      |         str = sprintf('%s\ntext(.5,.5,%s,%s)',str1,name,str2) ;
      |         set_param(blk,'MaskDisplay',str) ;
      |     end
      |     clear value1 value2 value3 value4 expr name1 name2 name3 name4 name fcn1 fcn2 fcn3 fcn4 str1 str2 str
      | 
      | else
      |     cellarr(5:8) = {'off'} ; val = get_param(blk,'MaskValues') ;
      |     for i=1:length(ind)
      |         a = findstr(val{ind(i)},'on') ;
      |         b(i) = isempty(a) ;
      |     end
      |     if isempty(find(b==0)) ;
      |         cellarr(ind) = {'on'} ;
      |     end
      | end
      | set_param(blk,'MaskVisibilities',cellarr) ;
      | clear blk value cellarr ind a b val i
      mask TypeOptions fromdens: Grams | Kilograms | Ounces | Pounds-Mass | Slugs
      mask Callback fromdens:
      | blk = gcb ;
      | value1 = get_param(blk,'fromdens') ;
      | value2 = get_param(blk,'perdens') ;
      | value3 = get_param(blk,'todens') ;
      | value4 = get_param(blk,'toperdens') ;
      | if strcmp(get_param(blk,'dens'),'on')
      |     switch value1
      |         case 'Grams'
      |             name1 = 'g/' ;
      |             fcn1  = 'u(1)*.001' ;
      |         case 'Kilograms'
      |             name1 = 'kg/' ;
      |             fcn1  = 'u(1)' ;
      |         case 'Ounces'
      |             name1 = 'oz/' ;
      |             fcn1  = 'u(1)*.45359237/16' ;
      |         case 'Pounds-Mass'
      |             name1 = 'lbm/' ;
      |             fcn1  = 'u(1)*.45359237' ;
      |         case 'Slugs'
      |             name1 = 'slg/' ;
      |             fcn1  = 'u(1)*14.5939';
      |     end
      |     switch value2
      |         case 'Milliliters'
      |             name2 = 'mL' ;
      |             fcn2  = '/(1e-6)' ;
      |         case 'Liters'
      |             name2 = 'L' ;
      |             fcn2  = '/.001' ;
      |         case 'Cubic Centimeters'
      |             name2 = 'cm^3' ;
      |             fcn2  = '/(1e-6)' ;
      |         case 'Cubic Meters'
      |             name2 = 'm^3' ;
      |             fcn2  = '' ;
      |         case 'Ounces'
      |             name2 = 'oz' ;
      |             fcn2  = '/(2.95735e-5)' ;
      |         case 'Gallons'
      |             name2 = 'gal' ;
      |             fcn2  = '/.0037854' ;
      |         case 'Cubic Inches'
      |             name2 = 'in^3' ;
      |             fcn2  = '/(1.6387e-5)' ;
      |         case 'Cubic Feet'
      |             name2 = 'ft^3' ;
      |             fcn2  = '/.02831685' ;
      |     end
      |     switch value3
      |         case 'Grams'
      |             name3 = 'g/' ;
      |             fcn3  = '/.001' ;
      |         case 'Kilograms'
      |             name3 = 'kg/' ;
      |             fcn3  = '' ;
      |         case 'Ounces'
      |             name3 = 'oz/' ;
      |             fcn3  = '/.45359237*16' ;
      |         case 'Pounds-Mass'
      |             name3 = 'lbm/' ;
      |             fcn3  = '/.45359237' ;
      |         case 'Slugs'
      |             name3 = 'slg/' ;
      |             fcn3  = '/14.5939';
      |     end
      |     switch value4
      |         case 'Milliliters'
      |             name4 = 'mL' ;
      |             fcn4  = '*(1e-6)' ;
      |         case 'Liters'
      |             name4 = 'L' ;
      |             fcn4  = '*.001' ;
      |         case 'Cubic Centimeters'
      |             name4 = 'cm^3' ;
      |             fcn4  = '*(1e-6)' ;
      |         case 'Cubic Meters'
      |             name4 = 'm^3' ;
      |             fcn4  = '' ;
      |         case 'Ounces'
      |             name4 = 'oz' ;
      |             fcn4  = '*(2.95735e-5)' ;
      |         case 'Gallons'
      |             name4 = 'gal' ;
      |             fcn4  = '*.0037854' ;
      |         case 'Cubic Inches'
      |             name4 = 'in^3' ;
      |             fcn4  = '*(1.6387e-5)' ;
      |         case 'Cubic Feet'
      |             name4 = 'ft^3' ;
      |             fcn4  = '*.02831685' ;
      |     end
      |     expr = [fcn1 fcn2 fcn3 fcn4] ;
      |     %set_param(blk,'func',func) ;
      |     set_param([blk '/conv_fcn'],'expr',expr) ;
      |     str1 = ['% this block of text is updated via dialog callbacks'];
      |     str2 = [char(39) 'horizontalAlignment' char(39) ',' char(39) 'center' char(39) ',' char(39) 'texmode' char(39) ',' char(39) 'on' char(39)] ;
      |     name = [char(39) name1 name2 ' to ' name3 name4 char(39)] ;
      |     str = sprintf('%s\ntext(.5,.5,%s,%s)',str1,name,str2) ;
      |     set_param(blk,'MaskDisplay',str) ;
      | end
      | clear blk value1 value2 value3 value4 expr name1 name2 name3 name4 name fcn1 fcn2 fcn3 fcn4 str1 str2 str
      mask TypeOptions perdens: Milliliters | Liters | Cubic Centimeters | Cubic Meters | Ounces | Gallons | Cubic Inches | Cubic Feet
      mask Callback perdens:
      | blk = gcb ;
      | value1 = get_param(blk,'fromdens') ;
      | value2 = get_param(blk,'perdens') ;
      | value3 = get_param(blk,'todens') ;
      | value4 = get_param(blk,'toperdens') ;
      | if strcmp(get_param(blk,'dens'),'on')
      |     switch value1
      |         case 'Grams'
      |             name1 = 'g/' ;
      |             fcn1  = 'u(1)*.001' ;
      |         case 'Kilograms'
      |             name1 = 'kg/' ;
      |             fcn1  = 'u(1)' ;
      |         case 'Ounces'
      |             name1 = 'oz/' ;
      |             fcn1  = 'u(1)*.45359237/16' ;
      |         case 'Pounds-Mass'
      |             name1 = 'lbm/' ;
      |             fcn1  = 'u(1)*.45359237' ;
      |         case 'Slugs'
      |             name1 = 'slg/' ;
      |             fcn1  = 'u(1)*14.5939';
      |     end
      |     switch value2
      |         case 'Milliliters'
      |             name2 = 'mL' ;
      |             fcn2  = '/(1e-6)' ;
      |         case 'Liters'
      |             name2 = 'L' ;
      |             fcn2  = '/.001' ;
      |         case 'Cubic Centimeters'
      |             name2 = 'cm^3' ;
      |             fcn2  = '/(1e-6)' ;
      |         case 'Cubic Meters'
      |             name2 = 'm^3' ;
      |             fcn2  = '' ;
      |         case 'Ounces'
      |             name2 = 'oz' ;
      |             fcn2  = '/(2.95735e-5)' ;
      |         case 'Gallons'
      |             name2 = 'gal' ;
      |             fcn2  = '/.0037854' ;
      |         case 'Cubic Inches'
      |             name2 = 'in^3' ;
      |             fcn2  = '/(1.6387e-5)' ;
      |         case 'Cubic Feet'
      |             name2 = 'ft^3' ;
      |             fcn2  = '/.02831685' ;
      |     end
      |     switch value3
      |         case 'Grams'
      |             name3 = 'g/' ;
      |             fcn3  = '/.001' ;
      |         case 'Kilograms'
      |             name3 = 'kg/' ;
      |             fcn3  = '' ;
      |         case 'Ounces'
      |             name3 = 'oz/' ;
      |             fcn3  = '/.45359237*16' ;
      |         case 'Pounds-Mass'
      |             name3 = 'lbm/' ;
      |             fcn3  = '/.45359237' ;
      |         case 'Slugs'
      |             name3 = 'slg/' ;
      |             fcn3  = '/14.5939';
      |     end
      |     switch value4
      |         case 'Milliliters'
      |             name4 = 'mL' ;
      |             fcn4  = '*(1e-6)' ;
      |         case 'Liters'
      |             name4 = 'L' ;
      |             fcn4  = '*.001' ;
      |         case 'Cubic Centimeters'
      |             name4 = 'cm^3' ;
      |             fcn4  = '*(1e-6)' ;
      |         case 'Cubic Meters'
      |             name4 = 'm^3' ;
      |             fcn4  = '' ;
      |         case 'Ounces'
      |             name4 = 'oz' ;
      |             fcn4  = '*(2.95735e-5)' ;
      |         case 'Gallons'
      |             name4 = 'gal' ;
      |             fcn4  = '*.0037854' ;
      |         case 'Cubic Inches'
      |             name4 = 'in^3' ;
      |             fcn4  = '*(1.6387e-5)' ;
      |         case 'Cubic Feet'
      |             name4 = 'ft^3' ;
      |             fcn4  = '*.02831685' ;
      |     end
      |     expr = [fcn1 fcn2 fcn3 fcn4] ;
      |     %set_param(blk,'func',func) ;
      |     set_param([blk '/conv_fcn'],'expr',expr) ;
      |     str1 = ['% this block of text is updated via dialog callbacks'];
      |     str2 = [char(39) 'horizontalAlignment' char(39) ',' char(39) 'center' char(39) ',' char(39) 'texmode' char(39) ',' char(39) 'on' char(39)] ;
      |     name = [char(39) name1 name2 ' to ' name3 name4 char(39)] ;
      |     str = sprintf('%s\ntext(.5,.5,%s,%s)',str1,name,str2) ;
      |     set_param(blk,'MaskDisplay',str) ;
      | end
      | clear blk value1 value2 value3 value4 expr name1 name2 name3 name4 name fcn1 fcn2 fcn3 fcn4 str1 str2 str
      mask TypeOptions todens: Grams | Kilograms | Ounces | Pounds-Mass | Slugs
      mask Callback todens:
      | blk = gcb ;
      | value1 = get_param(blk,'fromdens') ;
      | value2 = get_param(blk,'perdens') ;
      | value3 = get_param(blk,'todens') ;
      | value4 = get_param(blk,'toperdens') ;
      | if strcmp(get_param(blk,'dens'),'on')
      |     switch value1
      |         case 'Grams'
      |             name1 = 'g/' ;
      |             fcn1  = 'u(1)*.001' ;
      |         case 'Kilograms'
      |             name1 = 'kg/' ;
      |             fcn1  = 'u(1)' ;
      |         case 'Ounces'
      |             name1 = 'oz/' ;
      |             fcn1  = 'u(1)*.45359237/16' ;
      |         case 'Pounds-Mass'
      |             name1 = 'lbm/' ;
      |             fcn1  = 'u(1)*.45359237' ;
      |         case 'Slugs'
      |             name1 = 'slg/' ;
      |             fcn1  = 'u(1)*14.5939';
      |     end
      |     switch value2
      |         case 'Milliliters'
      |             name2 = 'mL' ;
      |             fcn2  = '/(1e-6)' ;
      |         case 'Liters'
      |             name2 = 'L' ;
      |             fcn2  = '/.001' ;
      |         case 'Cubic Centimeters'
      |             name2 = 'cm^3';
      |             fcn2  = '/(1e-6)' ;
      |         case 'Cubic Meters'
      |             name2 = 'm^3' ;
      |             fcn2  = '' ;
      |         case 'Ounces'
      |             name2 = 'oz' ;
      |             fcn2  = '/(2.95735e-5)' ;
      |         case 'Gallons'
      |             name2 = 'gal' ;
      |             fcn2  = '/.0037854' ;
      |         case 'Cubic Inches'
      |             name2 = 'in^3' ;
      |             fcn2  = '/(1.6387e-5)' ;
      |         case 'Cubic Feet'
      |             name2 = 'ft^3' ;
      |             fcn2  = '/.02831685' ;
      |     end
      |     switch value3
      |         case 'Grams'
      |             name3 = 'g/' ;
      |             fcn3  = '/.001' ;
      |         case 'Kilograms'
      |             name3 = 'kg/' ;
      |             fcn3  = '' ;
      |         case 'Ounces'
      |             name3 = 'oz/' ;
      |             fcn3  = '/.45359237*16' ;
      |         case 'Pounds-Mass'
      |             name3 = 'lbm/' ;
      |             fcn3  = '/.45359237' ;
      |         case 'Slugs'
      |             name3 = 'slg/' ;
      |             fcn3  = '/14.5939';
      |     end
      |     switch value4
      |         case 'Milliliters'
      |             name4 = 'mL' ;
      |             fcn4  = '*(1e-6)' ;
      |         case 'Liters'
      |             name4 = 'L' ;
      |             fcn4  = '*.001' ;
      |         case 'Cubic Centimeters'
      |             name4 = 'cm^3' ;
      |             fcn4  = '*(1e-6)' ;
      |         case 'Cubic Meters'
      |             name4 = 'm^3' ;
      |             fcn4  = '' ;
      |         case 'Ounces'
      |             name4 = 'oz' ;
      |             fcn4  = '*(2.95735e-5)' ;
      |         case 'Gallons'
      |             name4 = 'gal' ;
      |             fcn4  = '*.0037854' ;
      |         case 'Cubic Inches'
      |             name4 = 'in^3' ;
      |             fcn4  = '*(1.6387e-5)' ;
      |         case 'Cubic Feet'
      |             name4 = 'ft^3' ;
      |             fcn4  = '*.02831685' ;
      |     end
      |     expr = [fcn1 fcn2 fcn3 fcn4] ;
      |     %set_param(blk,'func',func) ;
      |     set_param([blk '/conv_fcn'],'expr',expr) ;
      |     str1 = ['% this block of text is updated via dialog callbacks'];
      |     str2 = [char(39) 'horizontalAlignment' char(39) ',' char(39) 'center' char(39) ',' char(39) 'texmode' char(39) ',' char(39) 'on' char(39)] ;
      |     name = [char(39) name1 name2 ' to ' name3 name4 char(39)] ;
      |     str = sprintf('%s\ntext(.5,.5,%s,%s)',str1,name,str2) ;
      |     set_param(blk,'MaskDisplay',str) ;
      | end
      | clear blk value1 value2 value3 value4 expr name1 name2 name3 name4 name fcn1 fcn2 fcn3 fcn4 str1 str2 str
      mask TypeOptions toperdens: Milliliters | Liters | Cubic Centimeters | Cubic Meters | Ounces | Gallons | Cubic Inches | Cubic Feet
      mask Callback toperdens:
      | blk = gcb ;
      | value1 = get_param(blk,'fromdens') ;
      | value2 = get_param(blk,'perdens') ;
      | value3 = get_param(blk,'todens') ;
      | value4 = get_param(blk,'toperdens') ;
      | if strcmp(get_param(blk,'dens'),'on')
      |     switch value1
      |         case 'Grams'
      |             name1 = 'g/' ;
      |             fcn1  = 'u(1)*.001' ;
      |         case 'Kilograms'
      |             name1 = 'kg/' ;
      |             fcn1  = 'u(1)' ;
      |         case 'Ounces'
      |             name1 = 'oz/' ;
      |             fcn1  = 'u(1)*.45359237/16' ;
      |         case 'Pounds-Mass'
      |             name1 = 'lbm/' ;
      |             fcn1  = 'u(1)*.45359237' ;
      |         case 'Slugs'
      |             name1 = 'slg/' ;
      |             fcn1  = 'u(1)*14.5939';
      |     end
      |     switch value2
      |         case 'Milliliters'
      |             name2 = 'mL' ;
      |             fcn2  = '/(1e-6)' ;
      |         case 'Liters'
      |             name2 = 'L' ;
      |             fcn2  = '/.001' ;
      |         case 'Cubic Centimeters'
      |             name2 = 'cm^3' ;
      |             fcn2  = '/(1e-6)' ;
      |         case 'Cubic Meters'
      |             name2 = 'm^3' ;
      |             fcn2  = '' ;
      |         case 'Ounces'
      |             name2 = 'oz' ;
      |             fcn2  = '/(2.95735e-5)' ;
      |         case 'Gallons'
      |             name2 = 'gal' ;
      |             fcn2  = '/.0037854' ;
      |         case 'Cubic Inches'
      |             name2 = 'in^3' ;
      |             fcn2  = '/(1.6387e-5)' ;
      |         case 'Cubic Feet'
      |             name2 = 'ft^3' ;
      |             fcn2  = '/.02831685' ;
      |     end
      |     switch value3
      |         case 'Grams'
      |             name3 = 'g/' ;
      |             fcn3  = '/.001' ;
      |         case 'Kilograms'
      |             name3 = 'kg/' ;
      |             fcn3  = '' ;
      |         case 'Ounces'
      |             name3 = 'oz/' ;
      |             fcn3  = '/.45359237*16' ;
      |         case 'Pounds-Mass'
      |             name3 = 'lbm/' ;
      |             fcn3  = '/.45359237' ;
      |         case 'Slugs'
      |             name3 = 'slg/' ;
      |             fcn3  = '/14.5939';
      |     end
      |     switch value4
      |         case 'Milliliters'
      |             name4 = 'mL' ;
      |             fcn4  = '*(1e-6)' ;
      |         case 'Liters'
      |             name4 = 'L' ;
      |             fcn4  = '*.001' ;
      |         case 'Cubic Centimeters'
      |             name4 = 'cm^3' ;
      |             fcn4  = '*(1e-6)' ;
      |         case 'Cubic Meters'
      |             name4 = 'm^3' ;
      |             fcn4  = '' ;
      |         case 'Ounces'
      |             name4 = 'oz' ;
      |             fcn4  = '*(2.95735e-5)' ;
      |         case 'Gallons'
      |             name4 = 'gal' ;
      |             fcn4  = '*.0037854' ;
      |         case 'Cubic Inches'
      |             name4 = 'in^3' ;
      |             fcn4  = '*(1.6387e-5)' ;
      |         case 'Cubic Feet'
      |             name4 = 'ft^3' ;
      |             fcn4  = '*.02831685' ;
      |     end
      |     expr = [fcn1 fcn2 fcn3 fcn4] ;
      |     %set_param(blk,'func',func) ;
      |     set_param([blk '/conv_fcn'],'expr',expr) ;
      |     str1 = ['% this block of text is updated via dialog callbacks'];
      |     str2 = [char(39) 'horizontalAlignment' char(39) ',' char(39) 'center' char(39) ',' char(39) 'texmode' char(39) ',' char(39) 'on' char(39)] ;
      |     name = [char(39) name1 name2 ' to ' name3 name4 char(39)] ;
      |     str = sprintf('%s\ntext(.5,.5,%s,%s)',str1,name,str2) ;
      |     set_param(blk,'MaskDisplay',str) ;
      | end
      | clear blk value1 value2 value3 value4 expr name1 name2 name3 name4 name fcn1 fcn2 fcn3 fcn4 str1 str2 str
      mask Callback energy:
      | blk = gcb ;
      | value = get_param(blk,'energy') ;
      | cellarr = get_param(blk,'MaskVisibilities') ;
      | ind = [1 4 9 12 15 18 21 24 27 30 33 38 43] ;
      | if strcmp(value,'on')
      |     cellarr(ind) = {'off'} ; cellarr(9:11) = {'on'} ;
      |     value1 = get_param(blk,'fromenergy') ;
      |     value2 = get_param(blk,'toenergy') ;
      |     if strcmp(get_param(blk,'energy'),'on') ;
      |         switch value1
      |             case 'Joules'
      |                 name1 = 'J' ;
      |                 fcn1  = 'u(1)' ;
      |             case 'Btu'
      |                 name1 = 'Btu' ;
      |                 fcn1  = 'u(1)*1055.05585' ;
      |             case 'Calories'
      |                 name1 = 'Cal' ;
      |                 fcn1  = 'u(1)*4.1868' ;
      |             case 'Foot-Pound(force)'
      |                 name1 = 'ft-lbf' ;
      |                 fcn1  = 'u(1)*1.355818' ;
      |             case 'Kilowatt-hour'
      |                 name1 = 'kw-hr' ;
      |                 fcn1  = 'u(1)*(3.6e6)' ;
      |         end
      |         switch value2
      |             case 'Joules'
      |                 name2 = 'J' ;
      |                 fcn2  = '' ;
      |             case 'Btu'
      |                 name2 = 'Btu' ;
      |                 fcn2  = '/1055.05585' ;
      |             case 'Calories'
      |                 name2 = 'Cal' ;
      |                 fcn2  = '/4.1868' ;
      |             case 'Foot-Pound(force)'
      |                 name2 = 'ft-lbf' ;
      |                 fcn2  = '/1.355818' ;
      |             case 'Kilowatt-hour'
      |                 name2 = 'kw-hr' ;
      |                 fcn2  = '/(3.6e6)' ;
      |         end
      |         expr = [fcn1 fcn2] ;
      |         %set_param(blk,'func',func) ;
      |         set_param([blk '/conv_fcn'],'expr',expr) ;
      |         str1 = ['% this block of text is updated via dialog callbacks'];
      |         str2 = [char(39) 'horizontalAlignment' char(39) ',' char(39) 'center' char(39) ',' char(39) 'texmode' char(39) ',' char(39) 'on' char(39)] ;
      |         name = [char(39) name1 ' to ' name2 char(39)] ;
      |         str = sprintf('%s\ntext(.5,.5,%s,%s)',str1,name,str2) ;
      |         set_param(blk,'MaskDisplay',str) ;
      |     end
      |     clear value1 value2 expr name1 name2 name fcn1 fcn2 str1 str2 str
      | else
      |     cellarr(10:11) = {'off'} ; val = get_param(blk,'MaskValues') ;
      |     for i=1:length(ind)
      |         a = findstr(val{ind(i)},'on') ;
      |         b(i) = isempty(a) ;
      |     end
      |     if isempty(find(b==0)) ;
      |         cellarr(ind) = {'on'} ;
      |     end
      | end
      | set_param(blk,'MaskVisibilities',cellarr) ;
      | clear blk value cellarr ind a b val i
      mask TypeOptions fromenergy: Joules | Btu | Calories | Foot-Pound(force) | Kilowatt-hour
      mask Callback fromenergy:
      | blk = gcb ;
      | value1 = get_param(blk,'fromenergy') ;
      | value2 = get_param(blk,'toenergy') ;
      | if strcmp(get_param(blk,'energy'),'on') ;
      |     switch value1
      |         case 'Joules'
      |             name1 = 'J' ;
      |             fcn1  = 'u(1)' ;
      |         case 'Btu'
      |             name1 = 'Btu' ;
      |             fcn1  = 'u(1)*1055.05585' ;
      |         case 'Calories'
      |             name1 = 'Cal' ;
      |             fcn1  = 'u(1)*4.1868' ;
      |         case 'Foot-Pound(force)'
      |             name1 = 'ft-lbf' ;
      |             fcn1  = 'u(1)*1.355818' ;
      |         case 'Kilowatt-hour'
      |             name1 = 'kw-hr' ;
      |             fcn1  = 'u(1)*(3.6e6)' ;
      |     end
      |     switch value2
      |         case 'Joules'
      |             name2 = 'J' ;
      |             fcn2  = '' ;
      |         case 'Btu'
      |             name2 = 'Btu' ;
      |             fcn2  = '/1055.05585' ;
      |         case 'Calories'
      |             name2 = 'Cal' ;
      |             fcn2  = '/4.1868' ;
      |         case 'Foot-Pound(force)'
      |             name2 = 'ft-lbf' ;
      |             fcn2  = '/1.355818' ;
      |         case 'Kilowatt-hour'
      |             name2 = 'kw-hr' ;
      |             fcn2  = '/(3.6e6)' ;
      |     end
      |     expr = [fcn1 fcn2] ;
      |     %set_param(blk,'func',func) ;
      |     set_param([blk '/conv_fcn'],'expr',expr) ;
      |     str1 = ['% this block of text is updated via dialog callbacks'];
      |     str2 = [char(39) 'horizontalAlignment' char(39) ',' char(39) 'center' char(39) ',' char(39) 'texmode' char(39) ',' char(39) 'on' char(39)] ;
      |     name = [char(39) name1 ' to ' name2 char(39)] ;
      |     str = sprintf('%s\ntext(.5,.5,%s,%s)',str1,name,str2) ;
      |     set_param(blk,'MaskDisplay',str) ;
      | end
      |     clear blk value1 value2 expr name1 name2 name fcn1 fcn2 str1 str2 str
      mask TypeOptions toenergy: Joules | Btu | Calories | Foot-Pound(force) | Kilowatt-hour
      mask Callback toenergy:
      | blk = gcb ;
      | value1 = get_param(blk,'fromenergy') ;
      | value2 = get_param(blk,'toenergy') ;
      | if strcmp(get_param(blk,'energy'),'on') ;
      |     switch value1
      |         case 'Joules'
      |             name1 = 'J' ;
      |             fcn1  = 'u(1)' ;
      |         case 'Btu'
      |             name1 = 'Btu' ;
      |             fcn1  = 'u(1)*1055.05585' ;
      |         case 'Calories'
      |             name1 = 'Cal' ;
      |             fcn1  = 'u(1)*4.1868' ;
      |         case 'Foot-Pound(force)'
      |             name1 = 'ft-lbf' ;
      |             fcn1  = 'u(1)*1.355818' ;
      |         case 'Kilowatt-hour'
      |             name1 = 'kw-hr' ;
      |             fcn1  = 'u(1)*(3.6e6)' ;
      |     end
      |     switch value2
      |         case 'Joules'
      |             name2 = 'J' ;
      |             fcn2  = '' ;
      |         case 'Btu'
      |             name2 = 'Btu' ;
      |             fcn2  = '/1055.05585' ;
      |         case 'Calories'
      |             name2 = 'Cal' ;
      |             fcn2  = '/4.1868' ;
      |         case 'Foot-Pound(force)'
      |             name2 = 'ft-lbf' ;
      |             fcn2  = '/1.355818' ;
      |         case 'Kilowatt-hour'
      |             name2 = 'kw-hr' ;
      |             fcn2  = '/(3.6e6)' ;
      |     end
      |     expr = [fcn1 fcn2] ;
      |     %set_param(blk,'func',func) ;
      |     set_param([blk '/conv_fcn'],'expr',expr) ;
      |     str1 = ['% this block of text is updated via dialog callbacks'];
      |     str2 = [char(39) 'horizontalAlignment' char(39) ',' char(39) 'center' char(39) ',' char(39) 'texmode' char(39) ',' char(39) 'on' char(39)] ;
      |     name = [char(39) name1 ' to ' name2 char(39)] ;
      |     str = sprintf('%s\ntext(.5,.5,%s,%s)',str1,name,str2) ;
      |     set_param(blk,'MaskDisplay',str) ;
      | end
      |     clear blk value1 value2 expr name1 name2 name fcn1 fcn2 str1 str2 str
      mask Callback power:
      | blk = gcb ;
      | value = get_param(blk,'power') ;
      | cellarr = get_param(blk,'MaskVisibilities') ;
      | ind = [1 4 9 12 15 18 21 24 27 30 33 38 43] ;
      | if strcmp(value,'on')
      |     cellarr(ind) = {'off'} ; cellarr(12:14) = {'on'} ;
      |     value1 = get_param(blk,'frompower') ;
      |     value2 = get_param(blk,'topower') ;
      |     if strcmp(get_param(blk,'power'),'on') ;
      |         switch value1
      |             case 'Watts'
      |                 name1 = 'W' ;
      |                 fcn1  = 'u(1)' ;
      |             case 'Kilowatts'
      |                 name1 = 'kW' ;
      |                 fcn1  = 'u(1)*1000' ;
      |             case 'Btu/s'
      |                 name1 = 'Btu/s' ;
      |                 fcn1  = 'u(1)*1055.056' ;
      |             case 'Btu/min'
      |                 name1 = 'Btu/min' ;
      |                 fcn1  = 'u(1)*17.584264' ;
      |             case 'Btu/hr'
      |                 name1 = 'Btu/hr' ;
      |                 fcn1  = 'u(1)*.293071' ;
      |             case 'Horsepower'
      |                 name1 = 'hp' ;
      |                 fcn1  = 'u(1)*745.69987' ;
      |         end
      |         switch value2
      |             case 'Watts'
      |                 name2 = 'W' ;
      |                 fcn2  = '' ;
      |             case 'Kilowatts'
      |                 name2 = 'kW' ;
      |                 fcn2  = '/1000' ;
      |             case 'Btu/s'
      |                 name2 = 'Btu/s' ;
      |                 fcn2  = '/1055.056' ;
      |             case 'Btu/min'
      |                 name2 = 'Btu/min' ;
      |                 fcn2  = '/17.584264' ;
      |             case 'Btu/hr'
      |                 name2 = 'Btu/hr' ;
      |                 fcn2  = '/.293071' ;
      |             case 'Horsepower'
      |                 name2 = 'hp' ;
      |                 fcn2  = '/745.69987' ;
      |         end
      |         expr = [fcn1 fcn2] ;
      |         %set_param(blk,'func',func) ;
      |         set_param([blk '/conv_fcn'],'expr',expr) ;
      |         str1 = ['% this block of text is updated via dialog callbacks'];
      |         str2 = [char(39) 'horizontalAlignment' char(39) ',' char(39) 'center' char(39) ',' char(39) 'texmode' char(39) ',' char(39) 'on' char(39)] ;
      |         name = [char(39) name1 ' to ' name2 char(39)] ;
      |         str = sprintf('%s\ntext(.5,.5,%s,%s)',str1,name,str2) ;
      |         set_param(blk,'MaskDisplay',str) ;
      |     end
      |     clear value1 value2 expr name1 name2 name fcn1 fcn2 str1 str2 str
      | else
      |     cellarr(13:14) = {'off'} ; val = get_param(blk,'MaskValues') ;
      |     for i=1:length(ind)
      |         a = findstr(val{ind(i)},'on') ;
      |         b(i) = isempty(a) ;
      |     end
      |     if isempty(find(b==0)) ;
      |         cellarr(ind) = {'on'} ;
      |     end
      | end
      | 
      | set_param(blk,'MaskVisibilities',cellarr) ;
      | clear blk value cellarr ind a b val i
      mask TypeOptions frompower: Watts | Kilowatts | Btu/s | Btu/min | Btu/hr | Horsepower
      mask Callback frompower:
      | blk = gcb ;
      | value1 = get_param(blk,'frompower') ;
      | value2 = get_param(blk,'topower') ;
      | if strcmp(get_param(blk,'power'),'on') ;
      |     switch value1
      |         case 'Watts'
      |             name1 = 'W' ;
      |             fcn1  = 'u(1)' ;
      |         case 'Kilowatts'
      |             name1 = 'kW' ;
      |             fcn1  = 'u(1)*1000' ;
      |         case 'Btu/s'
      |             name1 = 'Btu/s' ;
      |             fcn1  = 'u(1)*1055.056' ;
      |         case 'Btu/min'
      |             name1 = 'Btu/min' ;
      |             fcn1  = 'u(1)*17.584264' ;
      |         case 'Btu/hr'
      |             name1 = 'Btu/hr' ;
      |             fcn1  = 'u(1)*.293071' ;
      |         case 'Horsepower'
      |             name1 = 'hp' ;
      |             fcn1  = 'u(1)*745.69987' ;
      |     end
      |     switch value2
      |         case 'Watts'
      |             name2 = 'W' ;
      |             fcn2  = '' ;
      |         case 'Kilowatts'
      |             name2 = 'kW' ;
      |             fcn2  = '/1000' ;
      |         case 'Btu/s'
      |             name2 = 'Btu/s' ;
      |             fcn2  = '/1055.056' ;
      |         case 'Btu/min'
      |             name2 = 'Btu/min' ;
      |             fcn2  = '/17.584264' ;
      |         case 'Btu/hr'
      |             name2 = 'Btu/hr' ;
      |             fcn2  = '/.293071' ;
      |         case 'Horsepower'
      |             name2 = 'hp' ;
      |             fcn2  = '/745.69987' ;
      |     end
      |     expr = [fcn1 fcn2] ;
      |     %set_param(blk,'func',func) ;
      |     set_param([blk '/conv_fcn'],'expr',expr) ;
      |     str1 = ['% this block of text is updated via dialog callbacks'];
      |     str2 = [char(39) 'horizontalAlignment' char(39) ',' char(39) 'center' char(39) ',' char(39) 'texmode' char(39) ',' char(39) 'on' char(39)] ;
      |     name = [char(39) name1 ' to ' name2 char(39)] ;
      |     str = sprintf('%s\ntext(.5,.5,%s,%s)',str1,name,str2) ;
      |     set_param(blk,'MaskDisplay',str) ;
      | end
      |     clear blk value1 value2 expr name1 name2 name fcn1 fcn2 str1 str2 str
      mask TypeOptions topower: Watts | Kilowatts | Btu/s | Btu/min | Btu/hr | Horsepower
      mask Callback topower:
      | blk = gcb ;
      | value1 = get_param(blk,'frompower') ;
      | value2 = get_param(blk,'topower') ;
      | if strcmp(get_param(blk,'power'),'on') ;
      |     switch value1
      |         case 'Watts'
      |             name1 = 'W' ;
      |             fcn1  = 'u(1)' ;
      |         case 'Kilowatts'
      |             name1 = 'kW' ;
      |             fcn1  = 'u(1)*1000' ;
      |         case 'Btu/s'
      |             name1 = 'Btu/s' ;
      |             fcn1  = 'u(1)*1055.056' ;
      |         case 'Btu/min'
      |             name1 = 'Btu/min' ;
      |             fcn1  = 'u(1)*17.584264' ;
      |         case 'Btu/hr'
      |             name1 = 'Btu/hr' ;
      |             fcn1  = 'u(1)*.293071' ;
      |         case 'Horsepower'
      |             name1 = 'hp' ;
      |             fcn1  = 'u(1)*745.69987' ;
      |     end
      |     switch value2
      |         case 'Watts'
      |             name2 = 'W' ;
      |             fcn2  = '' ;
      |         case 'Kilowatts'
      |             name2 = 'kW' ;
      |             fcn2  = '/1000' ;
      |         case 'Btu/s'
      |             name2 = 'Btu/s' ;
      |             fcn2  = '/1055.056' ;
      |         case 'Btu/min'
      |             name2 = 'Btu/min' ;
      |             fcn2  = '/17.584264' ;
      |         case 'Btu/hr'
      |             name2 = 'Btu/hr' ;
      |             fcn2  = '/.293071' ;
      |         case 'Horsepower'
      |             name2 = 'hp' ;
      |             fcn2  = '/745.69987' ;
      |     end
      |     expr = [fcn1 fcn2] ;
      |     %set_param(blk,'func',func) ;
      |     set_param([blk '/conv_fcn'],'expr',expr) ;
      |     str1 = ['% this block of text is updated via dialog callbacks'];
      |     str2 = [char(39) 'horizontalAlignment' char(39) ',' char(39) 'center' char(39) ',' char(39) 'texmode' char(39) ',' char(39) 'on' char(39)] ;
      |     name = [char(39) name1 ' to ' name2 char(39)] ;
      |     str = sprintf('%s\ntext(.5,.5,%s,%s)',str1,name,str2) ;
      |     set_param(blk,'MaskDisplay',str) ;
      | end
      |     clear blk value1 value2 expr name1 name2 name fcn1 fcn2 str1 str2 str
      mask Callback force:
      | blk = gcb ;
      | value = get_param(blk,'force') ;
      | cellarr = get_param(blk,'MaskVisibilities') ;
      | ind = [1 4 9 12 15 18 21 24 27 30 33 38 43] ;
      | if strcmp(value,'on')
      |     cellarr(ind) = {'off'} ; cellarr(15:17) = {'on'} ;
      |     value1 = get_param(blk,'fromforce') ;
      |     value2 = get_param(blk,'toforce') ;
      |     if strcmp(get_param(blk,'force'),'on') ;
      |         switch value1
      |             case 'Newtons'
      |                 name1 = 'N' ;
      |                 fcn1  = 'u(1)' ;
      |             case 'Dyne'
      |                 name1 = 'dyne' ;
      |                 fcn1  = 'u(1)*(1e-5)' ;
      |             case 'Kilogram-Force'
      |                 name1 = 'kgf' ;
      |                 fcn1  = 'u(1)*9.80665' ;
      |             case 'Ton-Force'
      |                 name1 = 'tonf' ;
      |                 fcn1  = 'u(1)*8896.44323052' ;
      |             case 'Pound-Force'
      |                 name1 = 'lbf' ;
      |                 fcn1  = 'u(1)*4.448221615' ;
      |         end
      |         switch value2
      |             case 'Newtons'
      |                 name2 = 'N' ;
      |                 fcn2  = '' ;
      |             case 'Dyne'
      |                 name2 = 'dyne' ;
      |                 fcn2  = '/(1e-5)' ;
      |             case 'Kilogram-Force'
      |                 name2 = 'kgf' ;
      |                 fcn2  = '/9.80665' ;
      |             case 'Ton-Force'
      |                 name2 = 'tonf' ;
      |                 fcn2  = '/8896.44323052' ;
      |             case 'Pound-Force'
      |                 name2 = 'lbf' ;
      |                 fcn2  = '/4.448221615' ;
      |         end
      |         expr = [fcn1 fcn2] ;
      |         %set_param(blk,'func',func) ;
      |         set_param([blk '/conv_fcn'],'expr',expr) ;
      |         str1 = ['% this block of text is updated via dialog callbacks'];
      |         str2 = [char(39) 'horizontalAlignment' char(39) ',' char(39) 'center' char(39) ',' char(39) 'texmode' char(39) ',' char(39) 'on' char(39)] ;
      |         name = [char(39) name1 ' to ' name2 char(39)] ;
      |         str = sprintf('%s\ntext(.5,.5,%s,%s)',str1,name,str2) ;
      |         set_param(blk,'MaskDisplay',str) ;
      |     end
      |     clear value1 value2 expr name1 name2 name fcn1 fcn2 str1 str2 str
      | else
      |     cellarr(16:17) = {'off'} ;  val = get_param(blk,'MaskValues') ;
      |     for i=1:length(ind)
      |         a = findstr(val{ind(i)},'on') ;
      |         b(i) = isempty(a) ;
      |     end
      |     if isempty(find(b==0)) ;
      |         cellarr(ind) = {'on'} ;
      |     end
      | end
      | set_param(blk,'MaskVisibilities',cellarr) ;
      | clear blk value cellarr ind a b val i
      mask TypeOptions fromforce: Newtons | Dyne | Kilogram-Force | Ton-Force | Pound-Force
      mask Callback fromforce:
      | blk = gcb ;
      | value1 = get_param(blk,'fromforce') ;
      | value2 = get_param(blk,'toforce') ;
      | if strcmp(get_param(blk,'force'),'on') ;
      |     switch value1
      |         case 'Newtons'
      |             name1 = 'N' ;
      |             fcn1  = 'u(1)' ;
      |         case 'Dyne'
      |             name1 = 'dyne' ;
      |             fcn1  = 'u(1)*(1e-5)' ;
      |         case 'Kilogram-Force'
      |             name1 = 'kgf' ;
      |             fcn1  = 'u(1)*9.80665' ;
      |         case 'Ton-Force'
      |             name1 = 'tonf' ;
      |             fcn1  = 'u(1)*8896.44323052' ;
      |         case 'Pound-Force'
      |             name1 = 'lbf' ;
      |             fcn1  = 'u(1)*4.448221615' ;
      |     end
      |     switch value2
      |         case 'Newtons'
      |             name2 = 'N' ;
      |             fcn2  = '' ;
      |         case 'Dyne'
      |             name2 = 'dyne' ;
      |             fcn2  = '/(1e-5)' ;
      |         case 'Kilogram-Force'
      |             name2 = 'kgf' ;
      |             fcn2  = '/9.80665' ;
      |         case 'Ton-Force'
      |             name2 = 'tonf' ;
      |             fcn2  = '/8896.44323052' ;
      |         case 'Pound-Force'
      |             name2 = 'lbf' ;
      |             fcn2  = '/4.448221615' ;
      |     end
      |     expr = [fcn1 fcn2] ;
      |     %set_param(blk,'func',func) ;
      |     set_param([blk '/conv_fcn'],'expr',expr) ;
      |     str1 = ['% this block of text is updated via dialog callbacks'];
      |     str2 = [char(39) 'horizontalAlignment' char(39) ',' char(39) 'center' char(39) ',' char(39) 'texmode' char(39) ',' char(39) 'on' char(39)] ;
      |     name = [char(39) name1 ' to ' name2 char(39)] ;
      |     str = sprintf('%s\ntext(.5,.5,%s,%s)',str1,name,str2) ;
      |     set_param(blk,'MaskDisplay',str) ;
      | end
      |     clear blk value1 value2 expr name1 name2 name fcn1 fcn2 str1 str2 str
      mask TypeOptions toforce: Newtons | Dyne | Kilogram-Force | Ton-Force | Pound-Force
      mask Callback toforce:
      | blk = gcb ;
      | value1 = get_param(blk,'fromforce') ;
      | value2 = get_param(blk,'toforce') ;
      | if strcmp(get_param(blk,'force'),'on') ;
      |     switch value1
      |         case 'Newtons'
      |             name1 = 'N' ;
      |             fcn1  = 'u(1)' ;
      |         case 'Dyne'
      |             name1 = 'dyne' ;
      |             fcn1  = 'u(1)*(1e-5)' ;
      |         case 'Kilogram-Force'
      |             name1 = 'kgf' ;
      |             fcn1  = 'u(1)*9.80665' ;
      |         case 'Ton-Force'
      |             name1 = 'tonf' ;
      |             fcn1  = 'u(1)*8896.44323052' ;
      |         case 'Pound-Force'
      |             name1 = 'lbf' ;
      |             fcn1  = 'u(1)*4.448221615' ;
      |     end
      |     switch value2
      |         case 'Newtons'
      |             name2 = 'N' ;
      |             fcn2  = '' ;
      |         case 'Dyne'
      |             name2 = 'dyne' ;
      |             fcn2  = '/(1e-5)' ;
      |         case 'Kilogram-Force'
      |             name2 = 'kgf' ;
      |             fcn2  = '/9.80665' ;
      |         case 'Ton-Force'
      |             name2 = 'tonf' ;
      |             fcn2  = '/8896.44323052' ;
      |         case 'Pound-Force'
      |             name2 = 'lbf' ;
      |             fcn2  = '/4.448221615' ;
      |     end
      |     expr = [fcn1 fcn2] ;
      |     %set_param(blk,'func',func) ;
      |     set_param([blk '/conv_fcn'],'expr',expr) ;
      |     str1 = ['% this block of text is updated via dialog callbacks'];
      |     str2 = [char(39) 'horizontalAlignment' char(39) ',' char(39) 'center' char(39) ',' char(39) 'texmode' char(39) ',' char(39) 'on' char(39)] ;
      |     name = [char(39) name1 ' to ' name2 char(39)] ;
      |     str = sprintf('%s\ntext(.5,.5,%s,%s)',str1,name,str2) ;
      |     set_param(blk,'MaskDisplay',str) ;
      | end
      |     clear blk value1 value2 expr name1 name2 name fcn1 fcn2 str1 str2 str
      mask Callback temp:
      | blk = gcb ;
      | value = get_param(blk,'temp') ;
      | cellarr = get_param(blk,'MaskVisibilities') ;
      | ind = [1 4 9 12 15 18 21 24 27 30 33 38 43] ;
      | if strcmp(value,'on')
      |     cellarr(ind) = {'off'} ; cellarr(18:20) = {'on'} ;
      |     value1 = get_param(blk,'fromtemp') ;
      |     value2 = get_param(blk,'totemp') ;
      | 
      |     switch value1
      |         case 'Celcius'
      |             name1 = '{\circC}' ;
      |             fcn1  = '(u(1)+273.15)' ;
      |         case 'Kelvin'
      |             name1 = '{\circK}' ;
      |             fcn1  = 'u(1)' ;
      |         case 'Fahrenheit'
      |             name1 = '{\circF}' ;
      |             fcn1  = '(u(1)+459.67)/1.8' ;
      |         case 'Rankine'
      |             name1 = '{\circR}' ;
      |             fcn1  = 'u(1)/1.8' ;
      |     end
      |     switch value2
      |         case 'Celcius'
      |             name2 = '{\circC}' ;
      |             fcn2  = '-273.15'  ;
      |         case 'Kelvin'
      |             name2 = '{\circK}' ;
      |             fcn2  = '' ;
      |         case 'Fahrenheit'
      |             name2 = '{\circF}' ;
      |             fcn2  = '*1.8-459.67' ;
      |         case 'Rankine'
      |             name2 = '{\circR}' ;
      |             fcn2  = '*1.8' ;
      |     end
      |     expr = [fcn1 fcn2] ;
      |     %set_param(blk,'func',func) ;
      |     set_param([blk '/conv_fcn'],'expr',expr) ;
      |     str1 = ['% this block of text is updated via dialog callbacks'];
      |     str2 = [char(39) 'horizontalAlignment' char(39) ',' char(39) 'center' char(39) ',' char(39) 'texmode' char(39) ',' char(39) 'on' char(39)] ;
      |     name = [char(39) name1 ' to ' name2 char(39)] ;
      |     str = sprintf('%s\ntext(.5,.5,%s,%s)',str1,name,str2) ;
      |     set_param(blk,'MaskDisplay',str) ;
      |     clear value1 value2 expr name1 name2 name fcn1 fcn2 str1 str2 str
      | else
      |     cellarr(19:20) = {'off'} ; val = get_param(blk,'MaskValues') ;
      |     for i=1:length(ind)
      |         a = findstr(val{ind(i)},'on') ;
      |         b(i) = isempty(a) ;
      |     end
      |     if isempty(find(b==0)) ;
      |         cellarr(ind) = {'on'} ;
      |     end
      | end
      | set_param(blk,'MaskVisibilities',cellarr) ;
      | clear blk value cellarr ind a b val i
      mask TypeOptions fromtemp: Celcius | Kelvin | Fahrenheit | Rankine
      mask Callback fromtemp:
      | blk = gcb ;
      | value1 = get_param(blk,'fromtemp') ;
      | value2 = get_param(blk,'totemp') ;
      | if strcmp(get_param(blk,'temp'),'on') ;
      |     switch value1
      |         case 'Celcius'
      |             name1 = '{\circC}' ;
      |             fcn1  = '(u(1)+273.15)' ;
      |         case 'Kelvin'
      |             name1 = '{\circK}' ;
      |             fcn1  = 'u(1)' ;
      |         case 'Fahrenheit'
      |             name1 = '{\circF}' ;
      |             fcn1  = '(u(1)+459.67)/1.8' ;
      |         case 'Rankine'
      |             name1 = '{\circR}' ;
      |             fcn1  = 'u(1)/1.8' ;
      |     end
      |     switch value2
      |         case 'Celcius'
      |             name2 = '{\circC}' ;
      |             fcn2  = '-273.15'  ;
      |         case 'Kelvin'
      |             name2 = '{\circK}' ;
      |             fcn2  = '' ;
      |         case 'Fahrenheit'
      |             name2 = '{\circF}' ;
      |             fcn2  = '*1.8-459.67' ;
      |         case 'Rankine'
      |             name2 = '{\circR}' ;
      |             fcn2  = '*1.8' ;
      |     end
      |     expr = [fcn1 fcn2] ;
      |     %set_param(blk,'func',func) ;
      |     set_param([blk '/conv_fcn'],'expr',expr) ;
      |     str1 = ['% this block of text is updated via dialog callbacks'];
      |     str2 = [char(39) 'horizontalAlignment' char(39) ',' char(39) 'center' char(39) ',' char(39) 'texmode' char(39) ',' char(39) 'on' char(39)] ;
      |     name = [char(39) name1 ' to ' name2 char(39)] ;
      |     str = sprintf('%s\ntext(.5,.5,%s,%s)',str1,name,str2) ;
      |     set_param(blk,'MaskDisplay',str) ;
      | end
      |     clear blk value1 value2 expr name1 name2 name fcn1 fcn2 str1 str2 str
      mask TypeOptions totemp: Celcius | Kelvin | Fahrenheit | Rankine
      mask Callback totemp:
      | blk = gcb ;
      | value1 = get_param(blk,'fromtemp') ;
      | value2 = get_param(blk,'totemp') ;
      | if strcmp(get_param(blk,'temp'),'on') ;
      |     switch value1
      |         case 'Celcius'
      |             name1 = '{\circC}' ;
      |             fcn1  = '(u(1)+273.15)' ;
      |         case 'Kelvin'
      |             name1 = '{\circK}' ;
      |             fcn1  = 'u(1)' ;
      |         case 'Fahrenheit'
      |             name1 = '{\circF}' ;
      |             fcn1  = '(u(1)+459.67)/1.8' ;
      |         case 'Rankine'
      |             name1 = '{\circR}' ;
      |             fcn1  = 'u(1)/1.8' ;
      |     end
      |     switch value2
      |         case 'Celcius'
      |             name2 = '{\circC}' ;
      |             fcn2  = '-273.15'  ;
      |         case 'Kelvin'
      |             name2 = '{\circK}' ;
      |             fcn2  = '' ;
      |         case 'Fahrenheit'
      |             name2 = '{\circF}' ;
      |             fcn2  = '*1.8-459.67' ;
      |         case 'Rankine'
      |             name2 = '{\circR}' ;
      |             fcn2  = '*1.8' ;
      |     end
      |     expr = [fcn1 fcn2] ;
      |     %set_param(blk,'func',func) ;
      |     set_param([blk '/conv_fcn'],'expr',expr) ;
      |     str1 = ['% this block of text is updated via dialog callbacks'];
      |     str2 = [char(39) 'horizontalAlignment' char(39) ',' char(39) 'center' char(39) ',' char(39) 'texmode' char(39) ',' char(39) 'on' char(39)] ;
      |     name = [char(39) name1 ' to ' name2 char(39)] ;
      |     str = sprintf('%s\ntext(.5,.5,%s,%s)',str1,name,str2) ;
      |     set_param(blk,'MaskDisplay',str) ;
      | end
      |     clear blk value1 value2 expr name1 name2 name fcn1 fcn2 str1 str2 str
      mask Callback pres:
      | blk = gcb ;
      | value = get_param(blk,'pres') ;
      | cellarr = get_param(blk,'MaskVisibilities') ;
      | ind = [1 4 9 12 15 18 21 24 27 30 33 38 43] ;
      | if strcmp(value,'on') ;
      |     cellarr(ind) = {'off'} ; cellarr(21:23) = {'on'} ;
      |     value1 = get_param(blk,'frompres') ;
      |     value2 = get_param(blk,'topres') ;
      |     if strcmp(get_param(blk,'pres'),'on') ;
      |         switch value1
      |             case 'psia'
      |                 name1 = 'psia' ;
      |                 fcn1  = 'u(1)' ;
      |             case 'Pa'
      |                 name1 = 'Pa' ;
      |                 fcn1  = 'u(1)*(1.450377e-4)' ;
      |             case 'kPa'
      |                 name1 = 'kPa' ;
      |                 fcn1  = 'u(1)*(1.450377e-1)' ;
      |             case 'atm (0 C)'
      |                 name1 = 'atm' ;
      |                 fcn1  = 'u(1)*14.69595' ;
      |             case 'bar'
      |                 name1 = 'bar' ;
      |                 fcn1  = 'u(1)*14.503773773' ;
      |             case 'in Hg'
      |                 name1 = 'in Hg' ;
      |                 fcn1  = 'u(1)*.491154' ;
      |             case 'mm Hg'
      |                 name1 = 'mm Hg' ;
      |                 fcn1  = 'u(1)*.019336775' ;
      |             case 'in H20'
      |                 name1 = 'in H20' ;
      |                 fcn1  = 'u(1)*.036127292' ;
      |         end
      |         switch value2
      |             case 'psia'
      |                 name2 = 'psia' ;
      |                 fcn2  = '' ;
      |             case 'Pa'
      |                 name2 = 'Pa' ;
      |                 fcn2  = '/(1.450377e-4)' ;
      |             case 'kPa'
      |                 name2 = 'kPa' ;
      |                 fcn2  = '/(1.450377e-1)' ;
      |             case 'atm (0 C)'
      |                 name2 = 'atm' ;
      |                 fcn2  = '/14.69595' ;
      |             case 'bar'
      |                 name2 = 'bar' ;
      |                 fcn2  = '/14.503773773' ;
      |             case 'in Hg'
      |                 name2 = 'in Hg' ;
      |                 fcn2  = '/.491154' ;
      |             case 'mm Hg'
      |                 name2 = 'mm Hg' ;
      |                 fcn2  = '/.019336775' ;
      |             case 'in H20'
      |                 name2 = 'in H20' ;
      |                 fcn2  = '/.036127292' ;
      |         end
      |         expr = [fcn1 fcn2] ;
      |         %set_param(blk,'func',func) ;
      |         set_param([blk '/conv_fcn'],'expr',expr) ;
      |         str1 = ['% this block of text is updated via dialog callbacks'];
      |         str2 = [char(39) 'horizontalAlignment' char(39) ',' char(39) 'center' char(39) ',' char(39) 'texmode' char(39) ',' char(39) 'on' char(39)] ;
      |         name = [char(39) name1 ' to ' name2 char(39)] ;
      |         str = sprintf('%s\ntext(.5,.5,%s,%s)',str1,name,str2) ;
      |         set_param(blk,'MaskDisplay',str) ;
      |     end
      |     clear value1 value2 expr name1 name2 name fcn1 fcn2 str1 str2 str
      | else
      |     cellarr(22:23) = {'off'} ; val = get_param(blk,'MaskValues') ;
      |     for i=1:length(ind)
      |         a = findstr(val{ind(i)},'on') ;
      |         b(i) = isempty(a) ;
      |     end
      |     if isempty(find(b==0)) ;
      |         cellarr(ind) = {'on'} ;
      |     end
      | end
      | set_param(blk,'MaskVisibilities',cellarr) ;
      | clear blk value cellarr ind a b val i
      mask TypeOptions frompres: psia | Pa | kPa | atm (0 C) | bar | in Hg | mm Hg | in H20
      mask Callback frompres:
      | blk = gcb ;
      | value1 = get_param(blk,'frompres') ;
      | value2 = get_param(blk,'topres') ;
      | if strcmp(get_param(blk,'pres'),'on') ;
      |     switch value1
      |         case 'psia'
      |             name1 = 'psia' ;
      |             fcn1  = 'u(1)' ;
      |         case 'Pa'
      |             name1 = 'Pa' ;
      |             fcn1  = 'u(1)*(1.450377e-4)' ;
      |         case 'kPa'
      |             name1 = 'kPa' ;
      |             fcn1  = 'u(1)*(1.450377e-1)' ;
      |         case 'atm (0 C)'
      |             name1 = 'atm' ;
      |             fcn1  = 'u(1)*14.69595' ;
      |         case 'bar'
      |             name1 = 'bar' ;
      |             fcn1  = 'u(1)*14.503773773' ;
      |         case 'in Hg'
      |             name1 = 'in Hg' ;
      |             fcn1  = 'u(1)*.491154' ;
      |         case 'mm Hg'
      |             name1 = 'mm Hg' ;
      |             fcn1  = 'u(1)*.019336775' ;
      |         case 'in H20'
      |             name1 = 'in H20' ;
      |             fcn1  = 'u(1)*.036127292' ;
      |     end
      |     switch value2
      |         case 'psia'
      |             name2 = 'psia' ;
      |             fcn2  = '' ;
      |         case 'Pa'
      |             name2 = 'Pa' ;
      |             fcn2  = '/(1.450377e-4)' ;
      |         case 'kPa'
      |             name2 = 'kPa' ;
      |             fcn2  = '/(1.450377e-1)' ;
      |         case 'atm (0 C)'
      |             name2 = 'atm' ;
      |             fcn2  = '/14.69595' ;
      |         case 'bar'
      |             name2 = 'bar' ;
      |             fcn2  = '/14.503773773' ;
      |         case 'in Hg'
      |             name2 = 'in Hg' ;
      |             fcn2  = '/.491154' ;
      |         case 'mm Hg'
      |             name2 = 'mm Hg' ;
      |             fcn2  = '/.019336775' ;
      |         case 'in H20'
      |             name2 = 'in H20' ;
      |             fcn2  = '/.036127292' ;
      |     end
      |     expr = [fcn1 fcn2] ;
      |     %set_param(blk,'func',func) ;
      |     set_param([blk '/conv_fcn'],'expr',expr) ;
      |     str1 = ['% this block of text is updated via dialog callbacks'];
      |     str2 = [char(39) 'horizontalAlignment' char(39) ',' char(39) 'center' char(39) ',' char(39) 'texmode' char(39) ',' char(39) 'on' char(39)] ;
      |     name = [char(39) name1 ' to ' name2 char(39)] ;
      |     str = sprintf('%s\ntext(.5,.5,%s,%s)',str1,name,str2) ;
      |     set_param(blk,'MaskDisplay',str) ;
      | end
      |     clear blk value1 value2 expr name1 name2 name fcn1 fcn2 str1 str2 str
      mask TypeOptions topres: psia | Pa | kPa | atm (0 C) | bar | in Hg | mm Hg | in H20
      mask Callback topres:
      | blk = gcb ;
      | value1 = get_param(blk,'frompres') ;
      | value2 = get_param(blk,'topres') ;
      | if strcmp(get_param(blk,'pres'),'on') ;
      |     switch value1
      |         case 'psia'
      |             name1 = 'psia' ;
      |             fcn1  = 'u(1)' ;
      |         case 'Pa'
      |             name1 = 'Pa' ;
      |             fcn1  = 'u(1)*(1.450377e-4)' ;
      |         case 'kPa'
      |             name1 = 'kPa' ;
      |             fcn1  = 'u(1)*(1.450377e-1)' ;
      |         case 'atm (0 C)'
      |             name1 = 'atm' ;
      |             fcn1  = 'u(1)*14.69595' ;
      |         case 'bar'
      |             name1 = 'bar' ;
      |             fcn1  = 'u(1)*14.503773773' ;
      |         case 'in Hg'
      |             name1 = 'in Hg' ;
      |             fcn1  = 'u(1)*.491154' ;
      |         case 'mm Hg'
      |             name1 = 'mm Hg' ;
      |             fcn1  = 'u(1)*.019336775' ;
      |         case 'in H20'
      |             name1 = 'in H20' ;
      |             fcn1  = 'u(1)*.036127292' ;
      |     end
      |     switch value2
      |         case 'psia'
      |             name2 = 'psia' ;
      |             fcn2  = '' ;
      |         case 'Pa'
      |             name2 = 'Pa' ;
      |             fcn2  = '/(1.450377e-4)' ;
      |         case 'kPa'
      |             name2 = 'kPa' ;
      |             fcn2  = '/(1.450377e-1)' ;
      |         case 'atm (0 C)'
      |             name2 = 'atm' ;
      |             fcn2  = '/14.69595' ;
      |         case 'bar'
      |             name2 = 'bar' ;
      |             fcn2  = '/14.503773773' ;
      |         case 'in Hg'
      |             name2 = 'in Hg' ;
      |             fcn2  = '/.491154' ;
      |         case 'mm Hg'
      |             name2 = 'mm Hg' ;
      |             fcn2  = '/.019336775' ;
      |         case 'in H20'
      |             name2 = 'in H20' ;
      |             fcn2  = '/.036127292' ;
      |     end
      |     expr = [fcn1 fcn2] ;
      |     %set_param(blk,'func',func) ;
      |     set_param([blk '/conv_fcn'],'expr',expr) ;
      |     str1 = ['% this block of text is updated via dialog callbacks'];
      |     str2 = [char(39) 'horizontalAlignment' char(39) ',' char(39) 'center' char(39) ',' char(39) 'texmode' char(39) ',' char(39) 'on' char(39)] ;
      |     name = [char(39) name1 ' to ' name2 char(39)] ;
      |     str = sprintf('%s\ntext(.5,.5,%s,%s)',str1,name,str2) ;
      |     set_param(blk,'MaskDisplay',str) ;
      | end
      |     clear blk value1 value2 expr name1 name2 name fcn1 fcn2 str1 str2 str
      mask Callback length:
      | blk = gcb ;
      | value = get_param(blk,'length') ;
      | cellarr = get_param(blk,'MaskVisibilities') ;
      | ind = [1 4 9 12 15 18 21 24 27 30 33 38 43] ;
      | if strcmp(value,'on')
      |     cellarr(ind) = {'off'} ; cellarr(24:26) = {'on'} ;
      |     value1 = get_param(blk,'fromlength') ;
      |     value2 = get_param(blk,'tolength') ;
      |     if strcmp(get_param(blk,'length'),'on') ;
      |         switch value1
      |             case 'Millimeters'
      |                 name1 = 'mm' ;
      |                 fcn1  = 'u(1)*.001' ;
      |             case 'Centimeters'
      |                 name1 = 'cm' ;
      |                 fcn1  = 'u(1)*.01' ;
      |             case 'Meters'
      |                 name1 = 'm' ;
      |                 fcn1  = 'u(1)' ;
      |             case 'Kilometers'
      |                 name1 = 'km' ;
      |                 fcn1  = 'u(1)/1000' ;
      |             case 'Inches'
      |                 name1 = 'in' ;
      |                 fcn1  = 'u(1)*.0254' ;
      |             case 'Feet'
      |                 name1 = 'ft' ;
      |                 fcn1  = 'u(1)*.3048' ;
      |             case 'Yards'
      |                 name1 = 'yd' ;
      |                 fcn1  = 'u(1)*.9144' ;
      |             case 'Miles'
      |                 name1 = 'mi' ;
      |                 fcn1  = 'u(1)*1609.344' ;
      |             case 'Nautical Miles'
      |                 name1 = 'nmi' ;
      |                 fcn1  = 'u(1)*1852' ;
      |         end
      |         switch value2
      |             case 'Millimeters'
      |                 name2 = 'mm' ;
      |                 fcn2  = '/.001' ;
      |             case 'Centimeters'
      |                 name2 = 'cm' ;
      |                 fcn2 = '/.01' ;
      |             case 'Meters'
      |                 name2 = 'm' ;
      |                 fcn2  = '' ;
      |             case 'Kilometers'
      |                 name2 = 'km' ;
      |                 fcn2  = '/1000' ;
      |             case 'Inches'
      |                 name2 = 'in' ;
      |                 fcn2  = '/.0254' ;
      |             case 'Feet'
      |                 name2 = 'ft' ;
      |                 fcn2  = '/.3048' ;
      |             case 'Yards'
      |                 name2 = 'yd' ;
      |                 fcn2  = '/.9144' ;
      |             case 'Miles'
      |                 name2 = 'mi' ;
      |                 fcn2  = '/1609.344' ;
      |             case 'Nautical Miles'
      |                 name2 = 'nmi' ;
      |                 fcn2  = '/1852' ;
      |         end
      |         expr = [fcn1 fcn2] ;
      |         %set_param(blk,'func',func) ;
      |         set_param([blk '/conv_fcn'],'expr',expr) ;
      |         str1 = ['% this block of text is updated via dialog callbacks'];
      |         str2 = [char(39) 'horizontalAlignment' char(39) ',' char(39) 'center' char(39) ',' char(39) 'texmode' char(39) ',' char(39) 'on' char(39)] ;
      |         name = [char(39) name1 ' to ' name2 char(39)] ;
      |         str = sprintf('%s\ntext(.5,.5,%s,%s)',str1,name,str2) ;
      |         set_param(blk,'MaskDisplay',str) ;
      |     end
      |     clear value1 value2 expr name1 name2 name fcn1 fcn2 str1 str2 str
      | else
      |     cellarr(25:26) = {'off'} ; val = get_param(blk,'MaskValues') ;
      |     for i=1:length(ind)
      |         a = findstr(val{ind(i)},'on') ;
      |         b(i) = isempty(a) ;
      |     end
      |     if isempty(find(b==0)) ;
      |         cellarr(ind) = {'on'} ;
      |     end
      | end
      | set_param(blk,'MaskVisibilities',cellarr) ;
      | clear blk value cellarr ind a b val i
      mask TypeOptions fromlength: Millimeters | Centimeters | Meters | Kilometers | Inches | Feet | Yards | Miles | Nautical Miles
      mask Callback fromlength:
      | blk = gcb ;
      | value1 = get_param(blk,'fromlength') ;
      | value2 = get_param(blk,'tolength') ;
      | if strcmp(get_param(blk,'length'),'on') ;
      |     switch value1
      |         case 'Millimeters'
      |             name1 = 'mm' ;
      |             fcn1  = 'u(1)*.001' ;
      |         case 'Centimeters'
      |             name1 = 'cm' ;
      |             fcn1  = 'u(1)*.01' ;
      |         case 'Meters'
      |             name1 = 'm' ;
      |             fcn1  = 'u(1)' ;
      |         case 'Kilometers'
      |             name1 = 'km' ;
      |             fcn1  = 'u(1)/1000' ;
      |         case 'Inches'
      |             name1 = 'in' ;
      |             fcn1  = 'u(1)*.0254' ;
      |         case 'Feet'
      |             name1 = 'ft' ;
      |             fcn1  = 'u(1)*.3048' ;
      |         case 'Yards'
      |             name1 = 'yd' ;
      |             fcn1  = 'u(1)*.9144' ;
      |         case 'Miles'
      |             name1 = 'mi' ;
      |             fcn1  = 'u(1)*1609.344' ;
      |         case 'Nautical Miles'
      |             name1 = 'nmi' ;
      |             fcn1  = 'u(1)*1852' ;
      |     end
      |     switch value2
      |         case 'Millimeters'
      |             name2 = 'mm' ;
      |             fcn2  = '/.001' ;
      |         case 'Centimeters'
      |             name2 = 'cm' ;
      |             fcn2 = '/.01' ;
      |         case 'Meters'
      |             name2 = 'm' ;
      |             fcn2  = '' ;
      |         case 'Kilometers'
      |             name2 = 'km' ;
      |             fcn2  = '/1000' ;
      |         case 'Inches'
      |             name2 = 'in' ;
      |             fcn2  = '/.0254' ;
      |         case 'Feet'
      |             name2 = 'ft' ;
      |             fcn2  = '/.3048' ;
      |         case 'Yards'
      |             name2 = 'yd' ;
      |             fcn2  = '/.9144' ;
      |         case 'Miles'
      |             name2 = 'mi' ;
      |             fcn2  = '/1609.344' ;
      |         case 'Nautical Miles'
      |             name2 = 'nmi' ;
      |             fcn2  = '/1852' ;
      |     end
      |     expr = [fcn1 fcn2] ;
      |     %set_param(blk,'func',func) ;
      |     set_param([blk '/conv_fcn'],'expr',expr) ;
      |     str1 = ['% this block of text is updated via dialog callbacks'];
      |     str2 = [char(39) 'horizontalAlignment' char(39) ',' char(39) 'center' char(39) ',' char(39) 'texmode' char(39) ',' char(39) 'on' char(39)] ;
      |     name = [char(39) name1 ' to ' name2 char(39)] ;
      |     str = sprintf('%s\ntext(.5,.5,%s,%s)',str1,name,str2) ;
      |     set_param(blk,'MaskDisplay',str) ;
      | end
      | clear blk value1 value2 expr name1 name2 name fcn1 fcn2 str1 str2 str
      mask TypeOptions tolength: Millimeters | Centimeters | Meters | Kilometers | Inches | Feet | Yards | Miles | Nautical Miles
      mask Callback tolength:
      | blk = gcb ;
      | value1 = get_param(blk,'fromlength') ;
      | value2 = get_param(blk,'tolength') ;
      | if strcmp(get_param(blk,'length'),'on') ;
      |     switch value1
      |         case 'Millimeters'
      |             name1 = 'mm' ;
      |             fcn1  = 'u(1)*.001' ;
      |         case 'Centimeters'
      |             name1 = 'cm' ;
      |             fcn1  = 'u(1)*.01' ;
      |         case 'Meters'
      |             name1 = 'm' ;
      |             fcn1  = 'u(1)' ;
      |         case 'Kilometers'
      |             name1 = 'km' ;
      |             fcn1  = 'u(1)/1000' ;
      |         case 'Inches'
      |             name1 = 'in' ;
      |             fcn1  = 'u(1)*.0254' ;
      |         case 'Feet'
      |             name1 = 'ft' ;
      |             fcn1  = 'u(1)*.3048' ;
      |         case 'Yards'
      |             name1 = 'yd' ;
      |             fcn1  = 'u(1)*.9144' ;
      |         case 'Miles'
      |             name1 = 'mi' ;
      |             fcn1  = 'u(1)*1609.344' ;
      |         case 'Nautical Miles'
      |             name1 = 'nmi' ;
      |             fcn1  = 'u(1)*1852' ;
      |     end
      |     switch value2
      |         case 'Millimeters'
      |             name2 = 'mm' ;
      |             fcn2  = '/.001' ;
      |         case 'Centimeters'
      |             name2 = 'cm' ;
      |             fcn2 = '/.01' ;
      |         case 'Meters'
      |             name2 = 'm' ;
      |             fcn2  = '' ;
      |         case 'Kilometers'
      |             name2 = 'km' ;
      |             fcn2  = '/1000' ;
      |         case 'Inches'
      |             name2 = 'in' ;
      |             fcn2  = '/.0254' ;
      |         case 'Feet'
      |             name2 = 'ft' ;
      |             fcn2  = '/.3048' ;
      |         case 'Yards'
      |             name2 = 'yd' ;
      |             fcn2  = '/.9144' ;
      |         case 'Miles'
      |             name2 = 'mi' ;
      |             fcn2  = '/1609.344' ;
      |         case 'Nautical Miles'
      |             name2 = 'nmi' ;
      |             fcn2  = '/1852' ;
      |     end
      |     expr = [fcn1 fcn2] ;
      |     %set_param(blk,'func',func) ;
      |     set_param([blk '/conv_fcn'],'expr',expr) ;
      |     str1 = ['% this block of text is updated via dialog callbacks'];
      |     str2 = [char(39) 'horizontalAlignment' char(39) ',' char(39) 'center' char(39) ',' char(39) 'texmode' char(39) ',' char(39) 'on' char(39)] ;
      |     name = [char(39) name1 ' to ' name2 char(39)] ;
      |     str = sprintf('%s\ntext(.5,.5,%s,%s)',str1,name,str2) ;
      |     set_param(blk,'MaskDisplay',str) ;
      | end
      | clear blk value1 value2 expr name1 name2 name fcn1 fcn2 str1 str2 str
      mask Callback area:
      | blk = gcb ;
      | value = get_param(blk,'area') ;
      | cellarr = get_param(blk,'MaskVisibilities');
      | ind = [1 4 9 12 15 18 21 24 27 30 33 38 43] ;
      | if strcmp(value,'on')
      |     cellarr(ind) = {'off'} ; cellarr(27:29) = {'on'} ;
      |     value1 = get_param(blk,'fromarea') ;
      |     value2 = get_param(blk,'toarea') ;
      |     if strcmp(get_param(blk,'area'),'on') ;
      |         switch value1
      |             case 'Square Centimeters'
      |                 name1 = 'cm^2' ;
      |                 fcn1  = 'u(1)*(1e-4)' ;
      |             case 'Square Meters'
      |                 name1 = 'm^2' ;
      |                 fcn1  = 'u(1)' ;
      |             case 'Square Kilometers'
      |                 name1 = 'km^2' ;
      |                 fcn1  = 'u(1)*(1e6)' ;
      |             case 'Square Inches'
      |                 name1 = 'in^2' ;
      |                 fcn1  = 'u(1)*6.4516e-4' ;
      |             case 'Square Feet'
      |                 name1 = 'ft^2' ;
      |                 fcn1  = 'u(1)*.09290304' ;
      |             case 'Square Yards'
      |                 name1 = 'yd^2' ;
      |                 fcn1  = 'u(1)*.83612736' ;
      |             case 'Acres'
      |                 name1 = 'acre' ;
      |                 fcn1  = 'u(1)*4046.8564224' ;
      |             case 'Square Miles'
      |                 name1 = 'mi^2' ;
      |                 fcn1  = 'u(1)*(2.589988e6)' ;
      |         end
      |         switch value2
      |             case 'Square Centimeters'
      |                 name2 = 'cm^2' ;
      |                 fcn2  = '/(1e-4)' ;
      |             case 'Square Meters'
      |                 name2 = 'm^2' ;
      |                 fcn2  = '' ;
      |             case 'Square Kilometers'
      |                 name2 = 'km^2' ;
      |                 fcn2  = '/(1e6)' ;
      |             case 'Square Inches'
      |                 name2 = 'in^2' ;
      |                 fcn2  = '/6.4516e-4' ;
      |             case 'Square Feet'
      |                 name2 = 'ft^2' ;
      |                 fcn2  = '/.09290304' ;
      |             case 'Square Yards'
      |                 name2 = 'yd^2' ;
      |                 fcn2  = '/.83612736' ;
      |             case 'Acres'
      |                 name2 = 'acre' ;
      |                 fcn2  = '/4046.8564224' ;
      |             case 'Square Miles'
      |                 name2 = 'mi^2' ;
      |                 fcn2  = '/(2.589988e6)' ;
      |         end
      |         expr = [fcn1 fcn2] ;
      |         %set_param(blk,'func',func) ;
      |         set_param([blk '/conv_fcn'],'expr',expr) ;
      |         str1 = ['% this block of text is updated via dialog callbacks'];
      |         str2 = [char(39) 'horizontalAlignment' char(39) ',' char(39) 'center' char(39) ',' char(39) 'texmode' char(39) ',' char(39) 'on' char(39)] ;
      |         name = [char(39) name1 ' to ' name2 char(39)] ;
      |         str = sprintf('%s\ntext(.5,.5,%s,%s)',str1,name,str2) ;
      |         set_param(blk,'MaskDisplay',str) ;
      |     end
      |     clear value1 value2 expr name1 name2 name fcn1 fcn2 str1 str2 str
      | else
      |     cellarr(28:29) = {'off'} ; val = get_param(blk,'MaskValues') ;
      |     for i=1:length(ind)
      |         a = findstr(val{ind(i)},'on') ;
      |         b(i) = isempty(a) ;
      |     end
      |     if isempty(find(b==0)) ;
      |         cellarr(ind) = {'on'} ;
      |     end
      | end
      | set_param(blk,'MaskVisibilities',cellarr) ;
      | clear blk value cellarr ind a b val i
      mask TypeOptions fromarea: Square Centimeters | Square Meters | Square Kilometers | Square Inches | Square Feet | Square Yards | Acres | Square Miles
      mask Callback fromarea:
      | blk = gcb ;
      | value1 = get_param(blk,'fromarea') ;
      | value2 = get_param(blk,'toarea') ;
      | if strcmp(get_param(blk,'area'),'on') ;
      |     switch value1
      |         case 'Square Centimeters'
      |             name1 = 'cm^2' ;
      |             fcn1  = 'u(1)*(1e-4)' ;
      |         case 'Square Meters'
      |             name1 = 'm^2' ;
      |             fcn1  = 'u(1)' ;
      |         case 'Square Kilometers'
      |             name1 = 'km^2' ;
      |             fcn1  = 'u(1)*(1e6)' ;
      |         case 'Square Inches'
      |             name1 = 'in^2' ;
      |             fcn1  = 'u(1)*6.4516e-4' ;
      |         case 'Square Feet'
      |             name1 = 'ft^2' ;
      |             fcn1  = 'u(1)*.09290304' ;
      |         case 'Square Yards'
      |             name1 = 'yd^2' ;
      |             fcn1  = 'u(1)*.83612736' ;
      |         case 'Acres'
      |             name1 = 'acre' ;
      |             fcn1  = 'u(1)*4046.8564224' ;
      |         case 'Square Miles'
      |             name1 = 'mi^2' ;
      |             fcn1  = 'u(1)*(2.589988e6)' ;
      |     end
      |     switch value2
      |         case 'Square Centimeters'
      |             name2 = 'cm^2' ;
      |             fcn2  = '/(1e-4)' ;
      |         case 'Square Meters'
      |             name2 = 'm^2' ;
      |             fcn2  = '' ;
      |         case 'Square Kilometers'
      |             name2 = 'km^2' ;
      |             fcn2  = '/(1e6)' ;
      |         case 'Square Inches'
      |             name2 = 'in^2' ;
      |             fcn2  = '/6.4516e-4' ;
      |         case 'Square Feet'
      |             name2 = 'ft^2' ;
      |             fcn2  = '/.09290304' ;
      |         case 'Square Yards'
      |             name2 = 'yd^2' ;
      |             fcn2  = '/.83612736' ;
      |         case 'Acres'
      |             name2 = 'acre' ;
      |             fcn2  = '/4046.8564224' ;
      |         case 'Square Miles'
      |             name2 = 'mi^2' ;
      |             fcn2  = '/(2.589988e6)' ;
      |     end
      |     expr = [fcn1 fcn2] ;
      |     %set_param(blk,'func',func) ;
      |     set_param([blk '/conv_fcn'],'expr',expr) ;
      |     str1 = ['% this block of text is updated via dialog callbacks'];
      |     str2 = [char(39) 'horizontalAlignment' char(39) ',' char(39) 'center' char(39) ',' char(39) 'texmode' char(39) ',' char(39) 'on' char(39)] ;
      |     name = [char(39) name1 ' to ' name2 char(39)] ;
      |     str = sprintf('%s\ntext(.5,.5,%s,%s)',str1,name,str2) ;
      |     set_param(blk,'MaskDisplay',str) ;
      | end
      |     clear blk value1 value2 expr name1 name2 name fcn1 fcn2 str1 str2 str
      mask TypeOptions toarea: Square Centimeters | Square Meters | Square Kilometers | Square Inches | Square Feet | Square Yards | Acres | Square Miles
      mask Callback toarea:
      | blk = gcb ;
      | value1 = get_param(blk,'fromarea') ;
      | value2 = get_param(blk,'toarea') ;
      | if strcmp(get_param(blk,'area'),'on') ;
      |     switch value1
      |         case 'Square Centimeters'
      |             name1 = 'cm^2' ;
      |             fcn1  = 'u(1)*(1e-4)' ;
      |         case 'Square Meters'
      |             name1 = 'm^2' ;
      |             fcn1  = 'u(1)' ;
      |         case 'Square Kilometers'
      |             name1 = 'km^2' ;
      |             fcn1  = 'u(1)*(1e6)' ;
      |         case 'Square Inches'
      |             name1 = 'in^2' ;
      |             fcn1  = 'u(1)*6.4516e-4' ;
      |         case 'Square Feet'
      |             name1 = 'ft^2' ;
      |             fcn1  = 'u(1)*.09290304' ;
      |         case 'Square Yards'
      |             name1 = 'yd^2' ;
      |             fcn1  = 'u(1)*.83612736' ;
      |         case 'Acres'
      |             name1 = 'acre' ;
      |             fcn1  = 'u(1)*4046.8564224' ;
      |         case 'Square Miles'
      |             name1 = 'mi^2' ;
      |             fcn1  = 'u(1)*(2.589988e6)' ;
      |     end
      |     switch value2
      |         case 'Square Centimeters'
      |             name2 = 'cm^2' ;
      |             fcn2  = '/(1e-4)' ;
      |         case 'Square Meters'
      |             name2 = 'm^2' ;
      |             fcn2  = '' ;
      |         case 'Square Kilometers'
      |             name2 = 'km^2' ;
      |             fcn2  = '/(1e6)' ;
      |         case 'Square Inches'
      |             name2 = 'in^2' ;
      |             fcn2  = '/6.4516e-4' ;
      |         case 'Square Feet'
      |             name2 = 'ft^2' ;
      |             fcn2  = '/.09290304' ;
      |         case 'Square Yards'
      |             name2 = 'yd^2' ;
      |             fcn2  = '/.83612736' ;
      |         case 'Acres'
      |             name2 = 'acre' ;
      |             fcn2  = '/4046.8564224' ;
      |         case 'Square Miles'
      |             name2 = 'mi^2' ;
      |             fcn2  = '/(2.589988e6)' ;
      |     end
      |     expr = [fcn1 fcn2] ;
      |     %set_param(blk,'func',func) ;
      |     set_param([blk '/conv_fcn'],'expr',expr) ;
      |     str1 = ['% this block of text is updated via dialog callbacks'];
      |     str2 = [char(39) 'horizontalAlignment' char(39) ',' char(39) 'center' char(39) ',' char(39) 'texmode' char(39) ',' char(39) 'on' char(39)] ;
      |     name = [char(39) name1 ' to ' name2 char(39)] ;
      |     str = sprintf('%s\ntext(.5,.5,%s,%s)',str1,name,str2) ;
      |     set_param(blk,'MaskDisplay',str) ;
      | end
      |     clear blk value1 value2 expr name1 name2 name fcn1 fcn2 str1 str2 str
      mask Callback vol:
      | blk = gcb ;
      | value = get_param(blk,'vol') ;
      | cellarr = get_param(blk,'MaskVisibilities') ;
      | ind = [1 4 9 12 15 18 21 24 27 30 33 38 43] ;
      | if strcmp(value,'on') ;
      |     cellarr(ind) = {'off'} ; cellarr(30:32) = {'on'} ;
      |     value1 = get_param(blk,'fromvol') ;
      |     value2 = get_param(blk,'tovol') ;
      |     if strcmp(get_param(blk,'vol'),'on') ;
      |         switch value1
      |             case 'Milliliters'
      |                 name1 = 'mL' ;
      |                 fcn1  = 'u(1)*(1e-6)' ;
      |             case 'Liters'
      |                 name1 = 'L' ;
      |                 fcn1  = 'u(1)*.001' ;
      |             case 'Cubic Centimeters'
      |                 name1 = 'cm^3' ;
      |                 fcn1  = 'u(1)*(1e-6)' ;
      |             case 'Cubic Meters'
      |                 name1 = 'm^3' ;
      |                 fcn1  = 'u(1)' ;
      |             case 'Ounces'
      |                 name1 = 'oz' ;
      |                 fcn1  = 'u(1)*(2.95735e-5)' ;
      |             case 'Gallons'
      |                 name1 = 'gal' ;
      |                 fcn1  = 'u(1)*.0037854' ;
      |             case 'Cubic Inches'
      |                 name1 = 'in^3' ;
      |                 fcn1  = 'u(1)*(1.6387e-5)' ;
      |             case 'Cubic Feet'
      |                 name1 = 'ft^3' ;
      |                 fcn1  = 'u(1)*.02831685' ;
      |         end
      |         switch value2
      |             case 'Milliliters'
      |                 name2 = 'mL' ;
      |                 fcn2  = '/(1e-6)' ;
      |             case 'Liters'
      |                 name2 = 'L' ;
      |                 fcn2  = '/.001' ;
      |             case 'Cubic Centimeters'
      |                 name2 = 'cm^3' ;
      |                 fcn2  = '/(1e-6)' ;
      |             case 'Cubic Meters'
      |                 name2 = 'm^3' ;
      |                 fcn2  = '' ;
      |             case 'Ounces'
      |                 name2 = 'oz' ;
      |                 fcn2  = '/(2.95735e-5)' ;
      |             case 'Gallons'
      |                 name2 = 'gal' ;
      |                 fcn2  = '/.0037854' ;
      |             case 'Cubic Inches'
      |                 name2 = 'in^3' ;
      |                 fcn2  = '/(1.6387e-5)' ;
      |             case 'Cubic Feet'
      |                 name2 = 'ft^3' ;
      |                 fcn2  = '/.02831685' ;
      |         end
      |         expr = [fcn1 fcn2] ;
      |         %set_param(blk,'func',func) ;
      |         set_param([blk '/conv_fcn'],'expr',expr) ;
      |         str1 = ['% this block of text is updated via dialog callbacks'];
      |         str2 = [char(39) 'horizontalAlignment' char(39) ',' char(39) 'center' char(39) ',' char(39) 'texmode' char(39) ',' char(39) 'on' char(39)] ;
      |         name = [char(39) name1 ' to ' name2 char(39)] ;
      |         str = sprintf('%s\ntext(.5,.5,%s,%s)',str1,name,str2) ;
      |         set_param(blk,'MaskDisplay',str) ;
      |     end
      |     clear  value1 value2 expr name1 name2 name fcn1 fcn2 str1 str2 str
      | else
      |     cellarr(31:32) = {'off'} ; val = get_param(blk,'MaskValues') ;
      |     for i=1:length(ind)
      |         a = findstr(val{ind(i)},'on') ;
      |         b(i) = isempty(a) ;
      |     end
      |     if isempty(find(b==0)) ;
      |         cellarr(ind) = {'on'} ;
      |     end
      | end
      | set_param(blk,'MaskVisibilities',cellarr) ;
      | clear blk value cellarr ind a b val i
      mask TypeOptions fromvol: Milliliters | Liters | Cubic Centimeters | Cubic Meters | Ounces | Gallons | Cubic Inches | Cubic Feet
      mask Callback fromvol:
      | blk = gcb ;
      | value1 = get_param(blk,'fromvol') ;
      | value2 = get_param(blk,'tovol') ;
      | if strcmp(get_param(blk,'vol'),'on') ;
      |     switch value1
      |         case 'Milliliters'
      |             name1 = 'mL' ;
      |             fcn1  = 'u(1)*(1e-6)' ;
      |         case 'Liters'
      |             name1 = 'L' ;
      |             fcn1  = 'u(1)*.001' ;
      |         case 'Cubic Centimeters'
      |             name1 = 'cm^3' ;
      |             fcn1  = 'u(1)*(1e-6)' ;
      |         case 'Cubic Meters'
      |             name1 = 'm^3' ;
      |             fcn1  = 'u(1)' ;
      |         case 'Ounces'
      |             name1 = 'oz' ;
      |             fcn1  = 'u(1)*(2.95735e-5)' ;
      |         case 'Gallons'
      |             name1 = 'gal' ;
      |             fcn1  = 'u(1)*.0037854' ;
      |         case 'Cubic Inches'
      |             name1 = 'in^3' ;
      |             fcn1  = 'u(1)*(1.6387e-5)' ;
      |         case 'Cubic Feet'
      |             name1 = 'ft^3' ;
      |             fcn1  = 'u(1)*.02831685' ;
      |     end
      |     switch value2
      |         case 'Milliliters'
      |             name2 = 'mL' ;
      |             fcn2  = '/(1e-6)' ;
      |         case 'Liters'
      |             name2 = 'L' ;
      |             fcn2  = '/.001' ;
      |         case 'Cubic Centimeters'
      |             name2 = 'cm^3' ;
      |             fcn2  = '/(1e-6)' ;
      |         case 'Cubic Meters'
      |             name2 = 'm^3' ;
      |             fcn2  = '' ;
      |         case 'Ounces'
      |             name2 = 'oz' ;
      |             fcn2  = '/(2.95735e-5)' ;
      |         case 'Gallons'
      |             name2 = 'gal' ;
      |             fcn2  = '/.0037854' ;
      |         case 'Cubic Inches'
      |             name2 = 'in^3' ;
      |             fcn2  = '/(1.6387e-5)' ;
      |         case 'Cubic Feet'
      |             name2 = 'ft^3' ;
      |             fcn2  = '/.02831685' ;
      |     end
      |     expr = [fcn1 fcn2] ;
      |     %set_param(blk,'func',func) ;
      |     set_param([blk '/conv_fcn'],'expr',expr) ;
      |     str1 = ['% this block of text is updated via dialog callbacks'];
      |     str2 = [char(39) 'horizontalAlignment' char(39) ',' char(39) 'center' char(39) ',' char(39) 'texmode' char(39) ',' char(39) 'on' char(39)] ;
      |     name = [char(39) name1 ' to ' name2 char(39)] ;
      |     str = sprintf('%s\ntext(.5,.5,%s,%s)',str1,name,str2) ;
      |     set_param(blk,'MaskDisplay',str) ;
      | end
      |     clear blk value1 value2 expr name1 name2 name fcn1 fcn2 str1 str2 str
      mask TypeOptions tovol: Milliliters | Liters | Cubic Centimeters | Cubic Meters | Ounces | Gallons | Cubic Inches | Cubic Feet
      mask Callback tovol:
      | blk = gcb ;
      | value1 = get_param(blk,'fromvol') ;
      | value2 = get_param(blk,'tovol') ;
      | if strcmp(get_param(blk,'vol'),'on') ;
      |     switch value1
      |         case 'Milliliters'
      |             name1 = 'mL' ;
      |             fcn1  = 'u(1)*(1e-6)' ;
      |         case 'Liters'
      |             name1 = 'L' ;
      |             fcn1  = 'u(1)*.001' ;
      |         case 'Cubic Centimeters'
      |             name1 = 'cm^3' ;
      |             fcn1  = 'u(1)*(1e-6)' ;
      |         case 'Cubic Meters'
      |             name1 = 'm^3' ;
      |             fcn1  = 'u(1)' ;
      |         case 'Ounces'
      |             name1 = 'oz' ;
      |             fcn1  = 'u(1)*(2.95735e-5)' ;
      |         case 'Gallons'
      |             name1 = 'gal' ;
      |             fcn1  = 'u(1)*.0037854' ;
      |         case 'Cubic Inches'
      |             name1 = 'in^3' ;
      |             fcn1  = 'u(1)*(1.6387e-5)' ;
      |         case 'Cubic Feet'
      |             name1 = 'ft^3' ;
      |             fcn1  = 'u(1)*.02831685' ;
      |     end
      |     switch value2
      |         case 'Milliliters'
      |             name2 = 'mL' ;
      |             fcn2  = '/(1e-6)' ;
      |         case 'Liters'
      |             name2 = 'L' ;
      |             fcn2  = '/.001' ;
      |         case 'Cubic Centimeters'
      |             name2 = 'cm^3' ;
      |             fcn2  = '/(1e-6)' ;
      |         case 'Cubic Meters'
      |             name2 = 'm^3' ;
      |             fcn2  = '' ;
      |         case 'Ounces'
      |             name2 = 'oz' ;
      |             fcn2  = '/(2.95735e-5)' ;
      |         case 'Gallons'
      |             name2 = 'gal' ;
      |             fcn2  = '/.0037854' ;
      |         case 'Cubic Inches'
      |             name2 = 'in^3' ;
      |             fcn2  = '/(1.6387e-5)' ;
      |         case 'Cubic Feet'
      |             name2 = 'ft^3' ;
      |             fcn2  = '/.02831685' ;
      |     end
      |     expr = [fcn1 fcn2] ;
      |     %set_param(blk,'func',func) ;
      |     set_param([blk '/conv_fcn'],'expr',expr) ;
      |     str1 = ['% this block of text is updated via dialog callbacks'];
      |     str2 = [char(39) 'horizontalAlignment' char(39) ',' char(39) 'center' char(39) ',' char(39) 'texmode' char(39) ',' char(39) 'on' char(39)] ;
      |     name = [char(39) name1 ' to ' name2 char(39)] ;
      |     str = sprintf('%s\ntext(.5,.5,%s,%s)',str1,name,str2) ;
      |     set_param(blk,'MaskDisplay',str) ;
      | end
      |     clear blk value1 value2 expr name1 name2 name fcn1 fcn2 str1 str2 str
      mask Callback vel:
      | blk = gcb ;
      | value = get_param(blk,'vel') ;
      | cellarr = get_param(blk,'MaskVisibilities') ;
      | ind = [1 4 9 12 15 18 21 24 27 30 33 38 43] ;
